simulink model "Phase6__PHASE6_ASHUGANJ_CCPP_CLOSED_LOOP_TRIP"  (R2024a)
settings: Solver=FixedStepDiscrete  StartTime=0  StopTime=0.6  FixedStep=5e-05  RelTol=1e-3
PostLoadFcn:
  | p6startupdir=fileparts(get_param(bdroot,'FileName')); while ~isfile(fullfile(p6startupdir,'scripts','setup_phase6_workspace.m')), p6startupparent=fileparts(p6startupdir); assert(~strcmp(p6startupparent,p6startupdir),'Phase6:MissingScripts','Cannot locate the Phase6 scripts folder.'); p6startupdir=p6startupparent; end; addpath(fullfile(p6startupdir,'scripts')); setup_phase6_workspace; clear p6startupdir p6startupparent;
  | phase6_color_wires(bdroot);
model workspace (MAT data in the model file):
  C.Ts = 0.001
  C.droop = 0.05
  C.governorTime_s = 0.2
  C.turbineTime_s = 0.75
  C.avrGain = 200
  C.avrTime_s = 0.02
  C.fieldMin_pu = -5
  C.fieldMax_pu = 5
  C.powerMin_pu = 0
  C.powerMax_pu = 0.982532751092
  C.pm0 = 0.786549599338
  C.vf0 = 1.78657868075
  C.vref = 1
  C.breakerDelay_s = [0.05 0.05 0.05 0.05 0.05]
  C.source = 'Phase2 canonical academic governor/AVR assumptions; LF initial state; Phase6 assumed 50 ms breaker mechanism'
  D.dc_nominal_voltage_V = 110
  D.dc_cell_count = 55
  D.dc_capacity_Ah = 200
  D.dc_internal_resistance_ohm = 0.05
  D.dc_ocv_soc = [0 1]
  D.dc_ocv_V = [105 116]
  D.dc_soc_min = 0.2
  D.dc_soc_max = 1
  D.dc_soc_initial = 1
  D.dc_cutoff_voltage_V = 105
  D.dc_max_discharge_A = 200
  D.dc_max_charge_A = 40
  D.dc_charge_efficiency = 0.9
  D.charger_nominal_voltage_V = 110
  D.charger_rated_power_kW = 20
  D.charger_unit_count = 2
  D.charger_active_units = 1
  D.charger_efficiency = 0.925
  D.charger_float_voltage_V = 123.75
  D.charger_max_current_A = 180
  D.charger_min_current_A = 0
  D.charger_response_s = 0.1
  D.charger_voltage_gain_A_per_V = 50
  D.load_relay_kW = 0.3
  D.load_control_kW = 0.5
  D.load_instrumentation_kW = 0.4
  D.load_communications_kW = 0.2
  D.load_emergency_control_kW = 0.3
  D.load_excitation_electronics_kW = 0.7
  D.load_trip_kW = 2
  D.load_trip_duration_s = 0.2
  D.load_close_kW = 3
  D.load_close_duration_s = 0.5
  D.load_emergency_additional_kW = 5
  D.continuousLoad_W = 2400
  D.acPickup_pu = 0.8
  D.serviceTolerance_W = 1e-06
  D.provenance.canonicalValues = 2
  D.provenance.continuousLoad = 2
  D.provenance.acPickup = 3
  D.provenance.brownoutLoadEquivalent = 3
  D.provenance.idealBatteryCurrentLimiter = 3
  D.provenance.serviceTolerance = 3
  D.assumptions.chargerACPickup_pu = 0.8
  D.assumptions.brownoutResistiveLoad = 1
  D.assumptions.fullSOCChargeBlocking = 1
  D.assumptions.idealBatteryCurrentLimiting = 1
  D.assumptions.proportionalUnservedLoadAllocation = 1
  D.assumptions.settledInitialCharger = 1
  P : object (value not decoded)
  Phase6BuildInfo : object (value not decoded)
  Phase6LoadFlow.model = 'PHASE6_ASHUGANJ_CCPP_DYNAMIC_MODEL'
  Phase6LoadFlow.frequency = 50
  Phase6LoadFlow.basePower = 100000000
  Phase6LoadFlow.tolerance = 1e-07
  Phase6LoadFlow.Networks.busNumber = [1 2 3 4 5 6 7 8 9 10]
  Phase6LoadFlow.Networks.SwingBus = 4
  Phase6LoadFlow.status = 1
  Phase6LoadFlow.iterations = 4
  Phase6LoadFlow.error = ''
  Phase6LoadFlow.Ybus1 = [0.0873920462832-2.08170255025i  -0.0829764098408+1.99085235815i  0+0i  0+0i  -0.000264508037957+1.56595019834e-08i  0+0i  0+0i  0+0i  -0.00011499648785-6.81612243848e-09i  0+0i; -0.0829764098316+1.99085235807i  0.162493154937-4.08162124111i  0+0i  0+0i  0+0i  -1.21290815073+1.92736685493i  0+0i  0+0i  0+0i  0+0i; 0+0i  0+0i  48400.0004643-4.58000355417e-07i  0+0i  0+0i  -48400.0000058+2.3884238942e-07i  0+0i  0+0i  0+0i  0+0i; 0+0i  0+0i  0+0i  0.00750000727735-199.185842588i  0+0i  0+0i  0+0i  0+0i  0+0i  -0.00326087287198+86.6025402558i; -0.000264500119042-5.39692317404e-11i  0+0i  -4.60726984556e-06+6.85537528968e-06i  0+0i  2645001.51335-32.1863926658i  -16.4570656799+27.6603547922i  0+0i  0+0i  -1150000.47401+1.33105697926e-05i  0+0i; 0+0i  1.06269488092+2.01409326234i  -48400.000005-9.67689493729e-06i  0+0i  15.7260334296+28.0824148285i  48400.5136015-34.5657520976i  0+0i  0+0i  0+0i  0+0i; 0+0i  0+0i  0+0i  0+0i  0+0i  0+0i  263.293444669-1351.57295033i  0+0i  -131.646722331+675.78652439i  -131.646722335+675.786524392i; 0+0i  0+0i  0+0i  0+0i  0+0i  0+0i  0+0i  263.293444769-1351.57295033i  -131.646722308+675.786524358i  -131.646722335+675.786524392i; -0.000114999950295+1.06554793283e-11i  0+0i  0+0i  0+0i  -1150000.47401+1.7196895519e-05i  7.48164142323e-07-4.6186008574e-06i  -131.646722386+675.786524482i  -131.646722309+675.78652436i  500263.499587-1351.57295615i  0+0i; 0+0i  0+0i  0+0i  -0.00326087272452+86.6025402558i  0+0i  0+0i  -131.646722334+675.786524392i  -131.646722335+675.786524392i  0+0i  263.29486254-1389.22622871i]
  Phase6LoadFlow.bus(1).handle = NaN
  Phase6LoadFlow.bus(1).ID = '*1*'
  Phase6LoadFlow.bus(1).vbase = 230000
  Phase6LoadFlow.bus(1).vref = 1
  Phase6LoadFlow.bus(1).angle = 0
  Phase6LoadFlow.bus(1).sm = []
  Phase6LoadFlow.bus(1).asm = []
  Phase6LoadFlow.bus(1).vsrc = []
  Phase6LoadFlow.bus(1).pqload = []
  Phase6LoadFlow.bus(1).rlcload = []
  Phase6LoadFlow.bus(1).blocks = 122546.00293
  Phase6LoadFlow.bus(1).busType = 'PQ'
  Phase6LoadFlow.bus(1).Sref = 0
  Phase6LoadFlow.bus(1).Vbus = 0.95508394327+0.0629961905739i
  Phase6LoadFlow.bus(1).Sbus = 1.4977567369e-17-6.86106449339e-17i
  Phase6LoadFlow.bus(1).Sgen = 0
  Phase6LoadFlow.bus(1).Spqload = -1.4977567369e-17+6.86106449339e-17i
  Phase6LoadFlow.bus(1).Sshunt = 0.00369771783189+0.0832327500202i
  Phase6LoadFlow.bus(1).Qmin = -Inf
  Phase6LoadFlow.bus(1).Qmax = Inf
  Phase6LoadFlow.bus(1).QminReached = 0
  Phase6LoadFlow.bus(1).QmaxReached = 0
  Phase6LoadFlow.bus(2).handle = NaN
  Phase6LoadFlow.bus(2).ID = '*3*'
  Phase6LoadFlow.bus(2).vbase = 6600
  Phase6LoadFlow.bus(2).vref = 1
  Phase6LoadFlow.bus(2).angle = 0
  Phase6LoadFlow.bus(2).sm = []
  Phase6LoadFlow.bus(2).asm = []
  Phase6LoadFlow.bus(2).vsrc = []
  Phase6LoadFlow.bus(2).pqload = []
  Phase6LoadFlow.bus(2).rlcload = [1 2 3]
  Phase6LoadFlow.bus(2).blocks = [123416.003784 123430.003296 123438.003418]
  Phase6LoadFlow.bus(2).busType = 'PQ'
  Phase6LoadFlow.bus(2).Sref = -0.14-0.0867642073764i
  Phase6LoadFlow.bus(2).Vbus = 0.998654558552+0.0659079236223i
  Phase6LoadFlow.bus(2).Sbus = -0.14-0.0867642073764i
  Phase6LoadFlow.bus(2).Sgen = 0
  Phase6LoadFlow.bus(2).Spqload = 0.14+0.0867642073764i
  Phase6LoadFlow.bus(2).Sshunt = -0.00722084369742-0.185139717809i
  Phase6LoadFlow.bus(2).Qmin = -Inf
  Phase6LoadFlow.bus(2).Qmax = Inf
  Phase6LoadFlow.bus(2).QminReached = 0
  Phase6LoadFlow.bus(2).QmaxReached = 0
  Phase6LoadFlow.bus(3).handle = NaN
  Phase6LoadFlow.bus(3).ID = '*4*'
  Phase6LoadFlow.bus(3).vbase = 22000
  Phase6LoadFlow.bus(3).vref = 1
  Phase6LoadFlow.bus(3).angle = 0
  Phase6LoadFlow.bus(3).sm = 1
  Phase6LoadFlow.bus(3).asm = []
  Phase6LoadFlow.bus(3).vsrc = []
  Phase6LoadFlow.bus(3).pqload = []
  Phase6LoadFlow.bus(3).rlcload = 4
  Phase6LoadFlow.bus(3).blocks = [261.009277344 5832.00402832]
  Phase6LoadFlow.bus(3).busType = 'PV'
  Phase6LoadFlow.bus(3).Sref = 3.6
  Phase6LoadFlow.bus(3).Vbus = 0.92197936676-0.387239005356i
  Phase6LoadFlow.bus(3).Sbus = 3.6+0.276166455093i
  Phase6LoadFlow.bus(3).Sgen = 3.6+0.276166455093i
  Phase6LoadFlow.bus(3).Spqload = 0
  Phase6LoadFlow.bus(3).Sshunt = 0.000458423433884+5.17701742069e-06i
  Phase6LoadFlow.bus(3).Qmin = -Inf
  Phase6LoadFlow.bus(3).Qmax = Inf
  Phase6LoadFlow.bus(3).QminReached = 0
  Phase6LoadFlow.bus(3).QmaxReached = 0
  Phase6LoadFlow.bus(4).handle = NaN
  Phase6LoadFlow.bus(4).ID = '*5*'
  Phase6LoadFlow.bus(4).vbase = 230000
  Phase6LoadFlow.bus(4).vref = 1
  Phase6LoadFlow.bus(4).angle = 0
  Phase6LoadFlow.bus(4).sm = []
  Phase6LoadFlow.bus(4).asm = []
  Phase6LoadFlow.bus(4).vsrc = 1
  Phase6LoadFlow.bus(4).pqload = []
  Phase6LoadFlow.bus(4).rlcload = []
  Phase6LoadFlow.bus(4).blocks = 121606.003174
  Phase6LoadFlow.bus(4).busType = 'swing'
  Phase6LoadFlow.bus(4).Sref = 0
  Phase6LoadFlow.bus(4).Vbus = 1
  Phase6LoadFlow.bus(4).Sbus = -3.45133752941+0.264692642147i
  Phase6LoadFlow.bus(4).Sgen = -3.45133752941+0.264692642147i
  Phase6LoadFlow.bus(4).Spqload = 0
  Phase6LoadFlow.bus(4).Sshunt = 0.00423913447911+112.583302333i
  Phase6LoadFlow.bus(4).Qmin = -Inf
  Phase6LoadFlow.bus(4).Qmax = Inf
  Phase6LoadFlow.bus(4).QminReached = 0
  Phase6LoadFlow.bus(4).QmaxReached = 0
  Phase6LoadFlow.bus(5).handle = NaN
  Phase6LoadFlow.bus(5).ID = '*6*'
  Phase6LoadFlow.bus(5).vbase = 230000
  Phase6LoadFlow.bus(5).vref = 1
  Phase6LoadFlow.bus(5).angle = 0
  Phase6LoadFlow.bus(5).sm = []
  Phase6LoadFlow.bus(5).asm = []
  Phase6LoadFlow.bus(5).vsrc = []
  Phase6LoadFlow.bus(5).pqload = []
  Phase6LoadFlow.bus(5).rlcload = []
  Phase6LoadFlow.bus(5).blocks = 1170.01000977
  Phase6LoadFlow.bus(5).busType = 'PQ'
  Phase6LoadFlow.bus(5).Sref = 0
  Phase6LoadFlow.bus(5).Vbus = 0.998782663812+0.0182714556672i
  Phase6LoadFlow.bus(5).Sbus = 4.64828536298e-10+2.30425102224e-11i
  Phase6LoadFlow.bus(5).Sgen = 0
  Phase6LoadFlow.bus(5).Spqload = -4.64828536298e-10-2.30425102224e-11i
  Phase6LoadFlow.bus(5).Sshunt = 1491862.09587+0.00326094848941i
  Phase6LoadFlow.bus(5).Qmin = -Inf
  Phase6LoadFlow.bus(5).Qmax = Inf
  Phase6LoadFlow.bus(5).QminReached = 0
  Phase6LoadFlow.bus(5).QmaxReached = 0
  Phase6LoadFlow.bus(6).handle = NaN
  Phase6LoadFlow.bus(6).ID = '*8*'
  Phase6LoadFlow.bus(6).vbase = 22000
  Phase6LoadFlow.bus(6).vref = 1
  Phase6LoadFlow.bus(6).angle = 0
  Phase6LoadFlow.bus(6).sm = []
  Phase6LoadFlow.bus(6).asm = []
  Phase6LoadFlow.bus(6).vsrc = []
  Phase6LoadFlow.bus(6).pqload = []
  Phase6LoadFlow.bus(6).rlcload = []
  Phase6LoadFlow.bus(6).blocks = 122360.003052
  Phase6LoadFlow.bus(6).busType = 'PQ'
  Phase6LoadFlow.bus(6).Sref = 0
  Phase6LoadFlow.bus(6).Vbus = 0.921913008067-0.387204945387i
  Phase6LoadFlow.bus(6).Sbus = 8.11644335598e-12+5.36613214691e-13i
  Phase6LoadFlow.bus(6).Sgen = 0
  Phase6LoadFlow.bus(6).Spqload = -8.11644335598e-12-5.36613214691e-13i
  Phase6LoadFlow.bus(6).Sshunt = 0.00480844142117+0.107036142686i
  Phase6LoadFlow.bus(6).Qmin = -Inf
  Phase6LoadFlow.bus(6).Qmax = Inf
  Phase6LoadFlow.bus(6).QminReached = 0
  Phase6LoadFlow.bus(6).QmaxReached = 0
  Phase6LoadFlow.bus(7).handle = NaN
  Phase6LoadFlow.bus(7).ID = '*9*'
  Phase6LoadFlow.bus(7).vbase = 100000
  Phase6LoadFlow.bus(7).vref = 1
  Phase6LoadFlow.bus(7).angle = 0
  Phase6LoadFlow.bus(7).sm = []
  Phase6LoadFlow.bus(7).asm = []
  Phase6LoadFlow.bus(7).vsrc = []
  Phase6LoadFlow.bus(7).pqload = []
  Phase6LoadFlow.bus(7).rlcload = []
  Phase6LoadFlow.bus(7).blocks = 121211.00293
  Phase6LoadFlow.bus(7).busType = 'PQ'
  Phase6LoadFlow.bus(7).Sref = 0
  Phase6LoadFlow.bus(7).Vbus = 2.29707127118+0.0409383935568i
  Phase6LoadFlow.bus(7).Sbus = 5.31601850694e-13-5.12985224674e-13i
  Phase6LoadFlow.bus(7).Sgen = 0
  Phase6LoadFlow.bus(7).Spqload = -5.31601850694e-13+5.12985224674e-13i
  Phase6LoadFlow.bus(7).Sshunt = -7.7574979931e-08-0.000519611737109i
  Phase6LoadFlow.bus(7).Qmin = -Inf
  Phase6LoadFlow.bus(7).Qmax = Inf
  Phase6LoadFlow.bus(7).QminReached = 0
  Phase6LoadFlow.bus(7).QmaxReached = 0
  Phase6LoadFlow.bus(8).handle = NaN
  Phase6LoadFlow.bus(8).ID = '*10*'
  Phase6LoadFlow.bus(8).vbase = 100000
  Phase6LoadFlow.bus(8).vref = 1
  Phase6LoadFlow.bus(8).angle = 0
  Phase6LoadFlow.bus(8).sm = []
  Phase6LoadFlow.bus(8).asm = []
  Phase6LoadFlow.bus(8).vsrc = []
  Phase6LoadFlow.bus(8).pqload = []
  Phase6LoadFlow.bus(8).rlcload = []
  Phase6LoadFlow.bus(8).blocks = 120500.003662
  Phase6LoadFlow.bus(8).busType = 'PQ'
  Phase6LoadFlow.bus(8).Sref = 0
  Phase6LoadFlow.bus(8).Vbus = 2.29707127109+0.0409383933626i
  Phase6LoadFlow.bus(8).Sbus = -2.33221829935e-13-1.57153476947e-12i
  Phase6LoadFlow.bus(8).Sgen = 0
  Phase6LoadFlow.bus(8).Spqload = 2.33221829935e-13+1.57153476947e-12i
  Phase6LoadFlow.bus(8).Sshunt = 6.68020889729e-07-0.000519459230386i
  Phase6LoadFlow.bus(8).Qmin = -Inf
  Phase6LoadFlow.bus(8).Qmax = Inf
  Phase6LoadFlow.bus(8).QminReached = 0
  Phase6LoadFlow.bus(8).QmaxReached = 0
  Phase6LoadFlow.bus(9).handle = NaN
  Phase6LoadFlow.bus(9).ID = '*11*'
  Phase6LoadFlow.bus(9).vbase = 100000
  Phase6LoadFlow.bus(9).vref = 1
  Phase6LoadFlow.bus(9).angle = 0
  Phase6LoadFlow.bus(9).sm = []
  Phase6LoadFlow.bus(9).asm = []
  Phase6LoadFlow.bus(9).vsrc = []
  Phase6LoadFlow.bus(9).pqload = []
  Phase6LoadFlow.bus(9).rlcload = []
  Phase6LoadFlow.bus(9).blocks = 120500.003662
  Phase6LoadFlow.bus(9).busType = 'PQ'
  Phase6LoadFlow.bus(9).Sref = 0
  Phase6LoadFlow.bus(9).Vbus = 2.29719712563+0.0420241160697i
  Phase6LoadFlow.bus(9).Sbus = -5.34705002516e-10-1.81416564522e-11i
  Phase6LoadFlow.bus(9).Sgen = 0
  Phase6LoadFlow.bus(9).Spqload = 5.34705002516e-10+1.81416564522e-11i
  Phase6LoadFlow.bus(9).Sshunt = -3431273.84385-0.000545427580754i
  Phase6LoadFlow.bus(9).Qmin = -Inf
  Phase6LoadFlow.bus(9).Qmax = Inf
  Phase6LoadFlow.bus(9).QminReached = 0
  Phase6LoadFlow.bus(9).QmaxReached = 0
  Phase6LoadFlow.bus(10).handle = NaN
  Phase6LoadFlow.bus(10).ID = '*12*'
  Phase6LoadFlow.bus(10).vbase = 100000
  Phase6LoadFlow.bus(10).vref = 1
  Phase6LoadFlow.bus(10).angle = 0
  Phase6LoadFlow.bus(10).sm = []
  Phase6LoadFlow.bus(10).asm = []
  Phase6LoadFlow.bus(10).vsrc = []
  Phase6LoadFlow.bus(10).pqload = []
  Phase6LoadFlow.bus(10).rlcload = []
  Phase6LoadFlow.bus(10).blocks = 120508.003296
  Phase6LoadFlow.bus(10).busType = 'PQ'
  Phase6LoadFlow.bus(10).Sref = 0
  Phase6LoadFlow.bus(10).Vbus = 2.29694509322+0.0398527281134i
  Phase6LoadFlow.bus(10).Sbus = 2.61132424068e-12+4.5307306338e-14i
  Phase6LoadFlow.bus(10).Sgen = 0
  Phase6LoadFlow.bus(10).Spqload = -2.61132424068e-12-4.5307306338e-14i
  Phase6LoadFlow.bus(10).Sshunt = -0.00972652684513-258.332451941i
  Phase6LoadFlow.bus(10).Qmin = -Inf
  Phase6LoadFlow.bus(10).Qmax = Inf
  Phase6LoadFlow.bus(10).QminReached = 0
  Phase6LoadFlow.bus(10).QmaxReached = 0
  Phase6LoadFlow.sm.handle = 261.009277344
  Phase6LoadFlow.sm.busNumber = 3
  Phase6LoadFlow.sm.busID = '*4*'
  Phase6LoadFlow.sm.generatorType = 'PV'
  Phase6LoadFlow.sm.Pnom = 458000000
  Phase6LoadFlow.sm.Vnom = 22000
  Phase6LoadFlow.sm.P = 360000000
  Phase6LoadFlow.sm.Q = 0
  Phase6LoadFlow.sm.Qmin = -Inf
  Phase6LoadFlow.sm.Qmax = Inf
  Phase6LoadFlow.sm.S = 3.6+0.276166455093i
  Phase6LoadFlow.sm.I = 0.701350064837-0.359973841194i
  Phase6LoadFlow.sm.Pmec = 360239716.497
  Phase6LoadFlow.sm.Vt = 0.92197936676-0.387239005356i
  Phase6LoadFlow.sm.Vf = 1.78657868075
  Phase6LoadFlow.sm.th0 = -61.5748702309
  Phase6LoadFlow.sm.dw0 = 0
  Phase6LoadFlow.asm = []
  Phase6LoadFlow.vsrc.handle = 121606.003174
  Phase6LoadFlow.vsrc.busNumber = 4
  Phase6LoadFlow.vsrc.busID = '*5*'
  Phase6LoadFlow.vsrc.generatorType = 'swing'
  Phase6LoadFlow.vsrc.Vnom = 230000
  Phase6LoadFlow.vsrc.P = 10000
  Phase6LoadFlow.vsrc.Q = 0
  Phase6LoadFlow.vsrc.Qmin = -Inf
  Phase6LoadFlow.vsrc.Qmax = Inf
  Phase6LoadFlow.vsrc.S = -3.45133752941+0.264692642147i
  Phase6LoadFlow.vsrc.I = -3.45133752941-0.264692642147i
  Phase6LoadFlow.vsrc.Vt = 1
  Phase6LoadFlow.vsrc.Vint = 1
  Phase6LoadFlow.pqload = []
  Phase6LoadFlow.rlcload(1).handle = 123416.003784
  Phase6LoadFlow.rlcload(1).busNumber = 2
  Phase6LoadFlow.rlcload(1).busID = '*3*'
  Phase6LoadFlow.rlcload(1).loadType = 'PQ'
  Phase6LoadFlow.rlcload(1).Vnom = 6600
  Phase6LoadFlow.rlcload(1).P = 9017793.59431
  Phase6LoadFlow.rlcload(1).Q = 5588726.52496
  Phase6LoadFlow.rlcload(1).S = 0.0901779359431+0.0558872652496i
  Phase6LoadFlow.rlcload(1).I = 0.0935851574128-0.049786246322i
  Phase6LoadFlow.rlcload(1).Vt = 0.998654558552+0.0659079236223i
  Phase6LoadFlow.rlcload(2).handle = 123430.003296
  Phase6LoadFlow.rlcload(2).busNumber = 2
  Phase6LoadFlow.rlcload(2).busID = '*3*'
  Phase6LoadFlow.rlcload(2).loadType = 'PQ'
  Phase6LoadFlow.rlcload(2).Vnom = 6600
  Phase6LoadFlow.rlcload(2).P = 2491103.20285
  Phase6LoadFlow.rlcload(2).Q = 1543847.10634
  Phase6LoadFlow.rlcload(2).S = 0.0249110320285+0.0154384710634i
  Phase6LoadFlow.rlcload(2).I = 0.0258522534289-0.0137531067188i
  Phase6LoadFlow.rlcload(2).Vt = 0.998654558552+0.0659079236223i
  Phase6LoadFlow.rlcload(3).handle = 123438.003418
  Phase6LoadFlow.rlcload(3).busNumber = 2
  Phase6LoadFlow.rlcload(3).busID = '*3*'
  Phase6LoadFlow.rlcload(3).loadType = 'PQ'
  Phase6LoadFlow.rlcload(3).Vnom = 6600
  Phase6LoadFlow.rlcload(3).P = 2491103.20285
  Phase6LoadFlow.rlcload(3).Q = 1543847.10634
  Phase6LoadFlow.rlcload(3).S = 0.0249110320285+0.0154384710634i
  Phase6LoadFlow.rlcload(3).I = 0.0258522534289-0.0137531067188i
  Phase6LoadFlow.rlcload(3).Vt = 0.998654558552+0.0659079236223i
  Phase6LoadFlow.rlcload(4).handle = 5832.00402832
  Phase6LoadFlow.rlcload(4).busNumber = 3
  Phase6LoadFlow.rlcload(4).busID = '*4*'
  Phase6LoadFlow.rlcload(4).loadType = 'Z'
  Phase6LoadFlow.rlcload(4).Vnom = 22000
  Phase6LoadFlow.rlcload(4).P = 10
  Phase6LoadFlow.rlcload(4).Q = 0
  Phase6LoadFlow.rlcload(4).S = 1e-07
  Phase6LoadFlow.rlcload(4).I = 0
  Phase6LoadFlow.rlcload(4).Vt = 0.92197936676-0.387239005356i
  Phase6LoadFlow.LoadFlowSolver = 'PositiveSequence'
  Phase6Metadata.parameters.Ts = 0.001
  Phase6Metadata.parameters.droop = 0.05
  Phase6Metadata.parameters.governorTime_s = 0.2
  Phase6Metadata.parameters.turbineTime_s = 0.75
  Phase6Metadata.parameters.avrGain = 200
  Phase6Metadata.parameters.avrTime_s = 0.02
  Phase6Metadata.parameters.fieldMin_pu = -5
  Phase6Metadata.parameters.fieldMax_pu = 5
  Phase6Metadata.parameters.powerMin_pu = 0
  Phase6Metadata.parameters.powerMax_pu = 0.982532751092
  Phase6Metadata.parameters.pm0 = 0.786549599338
  Phase6Metadata.parameters.vf0 = 1.78657868075
  Phase6Metadata.parameters.vref = 1
  Phase6Metadata.parameters.breakerDelay_s = [0.05 0.05 0.05 0.05 0.05]
  Phase6Metadata.parameters.source = 'Phase2 canonical academic governor/AVR assumptions; LF initial state; Phase6 assumed 50 ms breaker mechanism'
  Phase6Metadata.relayParameters.settingValues = [17170.8  1.14472  15000  0.1  NaN  NaN; 4  0.2  20  0.15  NaN  NaN; 1380  0.8625  1600  0.55  NaN  NaN; 1500  0.9375  1600  0.8  NaN  NaN; 17171  1.14473333333  15000  NaN  3  NaN; 2403.8  0.160253333333  15000  NaN  NaN  0.045; 387.84  0.2424  1600  NaN  NaN  0.045; 320  0.2  1600  NaN  NaN  0.035; 320  0.2  1600  NaN  0.05  0.035]
  Phase6Metadata.relayParameters.settingSourceRows = [1 2 3 4 5 6 7 8 9]
  Phase6Metadata.relayParameters.pickup_A = [17170.8 1380 4 2403.8 387.84 320 320]
  Phase6Metadata.relayParameters.pickupSecondary_A = [1.14472 0.8625 0.2 0.160253333333 0.2424 0.2 0.2]
  Phase6Metadata.relayParameters.ctRatio = [15000 1600 20 15000 1600 1600 1600]
  Phase6Metadata.relayParameters.tms = [0.1 0.55 0.15]
  Phase6Metadata.relayParameters.delay_s = [0.045 0.045 0.035 0.035]
  Phase6Metadata.relayParameters.lvToHv = 0.095652173913
  Phase6Metadata.relayParameters.iecK = 0.14
  Phase6Metadata.relayParameters.iecAlpha = 0.02
  Phase6Metadata.relayParameters.highsetEnabled = [0 0 0 0 0 0 0]
  Phase6Metadata.relayParameters.slope1 = [0.3 0.3 0.3 0.3]
  Phase6Metadata.relayParameters.slope2 = [0.3 0.6 0.3 0.3]
  Phase6Metadata.relayParameters.knee_A = [12019 2585.6 1600 1600]
  Phase6Metadata.relayParameters.restraintFactor = 0.5
  Phase6Metadata.relayParameters.lineSchemeClearingProxy_s = 0.05
  Phase6Metadata.relayParameters.phase5.GEN_S_MVA = 458
  Phase6Metadata.relayParameters.phase5.GEN_V_kV = 22
  Phase6Metadata.relayParameters.phase5.GEN_rated_A = 12019
  Phase6Metadata.relayParameters.phase5.GEN_maximum_operating_A = 14309
  Phase6Metadata.relayParameters.phase5.GEN_phase_CT = 15000
  Phase6Metadata.relayParameters.phase5.GEN_51_pickup_A = 17170.8
  Phase6Metadata.relayParameters.phase5.GEN_51_secondary_A = 1.14472
  Phase6Metadata.relayParameters.phase5.GEN_51_TMS = 0.1
  Phase6Metadata.relayParameters.phase5.GEN_51N_CT = 20
  Phase6Metadata.relayParameters.phase5.GEN_51N_secondary_A = 0.2
  Phase6Metadata.relayParameters.phase5.GEN_51N_pickup_A = 4
  Phase6Metadata.relayParameters.phase5.GEN_51N_TMS = 0.15
  Phase6Metadata.relayParameters.phase5.GEN_87G_pu = 0.2
  Phase6Metadata.relayParameters.phase5.GEN_87G_pickup_A = 2403.8
  Phase6Metadata.relayParameters.phase5.GEN_87G_highset_enabled = 0
  Phase6Metadata.relayParameters.phase5.GEN_87G_time_s = 0.045
  Phase6Metadata.relayParameters.phase5.GEN_Xdpp_sat_pu = 0.2248
  Phase6Metadata.relayParameters.phase5.GEN_Xdpp_unsat_pu = 0.2608
  Phase6Metadata.relayParameters.phase5.GEN_X2_pu = 0.2242
  Phase6Metadata.relayParameters.phase5.GEN_X0_pu = 0.128
  Phase6Metadata.relayParameters.phase5.GEN_Ra_ohm = 0.00089
  Phase6Metadata.relayParameters.phase5.GEN_R1_pu = 0.000842190082645
  Phase6Metadata.relayParameters.phase5.GEN_R2_pu = 0.000842190082645
  Phase6Metadata.relayParameters.phase5.GEN_R0_pu = 0.00126328512397
  Phase6Metadata.relayParameters.phase5.GSUT_S_MVA = 515
  Phase6Metadata.relayParameters.phase5.GSUT_HV_kV = 230
  Phase6Metadata.relayParameters.phase5.GSUT_LV_kV = 22
  Phase6Metadata.relayParameters.phase5.GSUT_rated_exact_A = 1292.76255927
  Phase6Metadata.relayParameters.phase5.GSUT_rated_A = 1292.8
  Phase6Metadata.relayParameters.phase5.GSUT_maximum_load_anchor_A = 1149.68010126
  Phase6Metadata.relayParameters.phase5.GSUT_CT = 1600
  Phase6Metadata.relayParameters.phase5.GSUT_documentary_CT = 1500
  Phase6Metadata.relayParameters.phase5.GSUT_51_pickup_A = 1380
  Phase6Metadata.relayParameters.phase5.GSUT_51_secondary_A = 0.8625
  Phase6Metadata.relayParameters.phase5.GSUT_51_TMS = 0.55
  Phase6Metadata.relayParameters.phase5.GSUT_87T_pu = 0.3
  Phase6Metadata.relayParameters.phase5.GSUT_87T_pickup_A = 387.84
  Phase6Metadata.relayParameters.phase5.GSUT_87T_slope1_percent = 30
  Phase6Metadata.relayParameters.phase5.GSUT_87T_slope2_percent = 60
  Phase6Metadata.relayParameters.phase5.GSUT_87T_time_s = 0.045
  Phase6Metadata.relayParameters.phase5.GSUT_Z1_pu = 0.1663
  Phase6Metadata.relayParameters.phase5.GSUT_copper_loss_MW = 0.9122
  Phase6Metadata.relayParameters.phase5.GSUT_OEM_Z1_pu = 0.16
  Phase6Metadata.relayParameters.phase5.GSUT_OEM_copper_loss_MW = 1.095
  Phase6Metadata.relayParameters.phase5.GSUT_R1_pu = 0.00177126213592
  Phase6Metadata.relayParameters.phase5.GSUT_X1_pu = 0.166290566872
  Phase6Metadata.relayParameters.phase5.GSUT_vector_clock = 1
  Phase6Metadata.relayParameters.phase5.GSUT_HV_solid_grounded = 1
  Phase6Metadata.relayParameters.phase5.Q0_CT = 1600
  Phase6Metadata.relayParameters.phase5.Q0_51_pickup_A = 1500
  Phase6Metadata.relayParameters.phase5.Q0_51_secondary_A = 0.9375
  Phase6Metadata.relayParameters.phase5.Q0_51_TMS = 0.8
  Phase6Metadata.relayParameters.phase5.Q0_continuous_A = 2000
  Phase6Metadata.relayParameters.phase5.Q0_interrupting_kA = 50
  Phase6Metadata.relayParameters.phase5.Q0_making_kA = 125
  Phase6Metadata.relayParameters.phase5.Q0_shortcircuit_s = 3
  Phase6Metadata.relayParameters.phase5.BUS_87B_pu = 0.2
  Phase6Metadata.relayParameters.phase5.BUS_87B_base_A = 1600
  Phase6Metadata.relayParameters.phase5.BUS_87B_pickup_A = 320
  Phase6Metadata.relayParameters.phase5.BUS_87B_slope_percent = 30
  Phase6Metadata.relayParameters.phase5.BUS_87B_time_s = 0.035
  Phase6Metadata.relayParameters.phase5.LINE_87L_pu = 0.2
  Phase6Metadata.relayParameters.phase5.LINE_87L_base_A = 1600
  Phase6Metadata.relayParameters.phase5.LINE_87L_pickup_A = 320
  Phase6Metadata.relayParameters.phase5.LINE_87L_time_s = 0.035
  Phase6Metadata.relayParameters.phase5.LINE_87L_clearing_s = 0.05
  Phase6Metadata.relayParameters.phase5.BF_230kV_s = 0.15
  Phase6Metadata.relayParameters.phase5.BF_22kV_s = 0.12
  Phase6Metadata.relayParameters.phase5.CTI_s = 0.3
  Phase6Metadata.relayParameters.phase5.GEN_64G_U20min_V = 1
  Phase6Metadata.relayParameters.phase5.GEN_64G_I20min_A = 0.01
  Phase6Metadata.relayParameters.phase5.GEN_64G_trip_R_ohm = 20
  Phase6Metadata.relayParameters.phase5.GEN_64G_alarm_R_ohm = 100
  Phase6Metadata.relayParameters.phase5.GEN_64G_trip_delay_s = 1
  Phase6Metadata.relayParameters.phase5.GEN_64G_alarm_delay_s = 10
  Phase6Metadata.relayParameters.phase5.GEN_64G_correction_angle_deg = 0
  Phase6Metadata.relayParameters.phase5.NER_R_ohm = 60
  Phase6Metadata.relayParameters.phase5.NER_rating_kVA = 135
  Phase6Metadata.relayParameters.phase5.NER_duration_s = 20
  Phase6Metadata.relayParameters.phase5.NER_primary_kV = 12.7017059222
  Phase6Metadata.relayParameters.phase5.NER_secondary_V = 500
  Phase6Metadata.relayParameters.phase5.NGT_ratio = 25.4034118443
  Phase6Metadata.relayParameters.phase5.NER_loading_LV_ohm = 2.62
  Phase6Metadata.relayParameters.phase5.NER_effective_HV_ohm = 1750.77333333
  Phase6Metadata.relayParameters.phase5.SOUTH_length_km = 0.7
  Phase6Metadata.relayParameters.phase5.SOUTH_circuits = 2
  Phase6Metadata.relayParameters.phase5.SOUTH_R1_per_km = 0.08
  Phase6Metadata.relayParameters.phase5.SOUTH_R1_total_ohm = 0.056
  Phase6Metadata.relayParameters.phase5.SOUTH_X1_per_km = 0.35
  Phase6Metadata.relayParameters.phase5.SOUTH_X1_total_ohm = 0.245
  Phase6Metadata.relayParameters.phase5.SOUTH_B1_per_km = 4.2
  Phase6Metadata.relayParameters.phase5.SOUTH_B1_total_uS = 2.94
  Phase6Metadata.relayParameters.phase5.SOUTH_R0_per_km = 0.25
  Phase6Metadata.relayParameters.phase5.SOUTH_R0_total_ohm = 0.175
  Phase6Metadata.relayParameters.phase5.SOUTH_X0_per_km = 1.2
  Phase6Metadata.relayParameters.phase5.SOUTH_X0_total_ohm = 0.84
  Phase6Metadata.relayParameters.phase5.SOUTH_B0_per_km = 2.8
  Phase6Metadata.relayParameters.phase5.SOUTH_B0_total_uS = 1.96
  Phase6Metadata.relayParameters.phase5.DIST21_zone1_fraction = 0.8
  Phase6Metadata.relayParameters.phase5.DIST21_zone1_R_ohm = 0.0448
  Phase6Metadata.relayParameters.phase5.DIST21_zone1_X_ohm = 0.196
  Phase6Metadata.relayParameters.phase5.DIST21_zone1_time_s = 0
  Phase6Metadata.relayParameters.phase5.DIST21_zone2_fraction = 1.2
  Phase6Metadata.relayParameters.phase5.DIST21_zone2_R_ohm = 0.0672
  Phase6Metadata.relayParameters.phase5.DIST21_zone2_X_ohm = 0.294
  Phase6Metadata.relayParameters.phase5.DIST21_zone2_time_s = 0.3
  Phase6Metadata.relayParameters.phase5.DIST21_zone3_fraction = 2
  Phase6Metadata.relayParameters.phase5.DIST21_zone3_R_ohm = 0.112
  Phase6Metadata.relayParameters.phase5.DIST21_zone3_X_ohm = 0.49
  Phase6Metadata.relayParameters.phase5.DIST21_zone3_time_s = 0.8
  Phase6Metadata.relayParameters.phase5.NORTH_BHULTA_length_km = 69
  Phase6Metadata.relayParameters.phase5.NORTH_BHULTA_circuits = 2
  Phase6Metadata.relayParameters.phase5.NORTH_BHULTA_voltage_kV = 400
  Phase6Metadata.relayParameters.phase5.NORTH_BHULTA_R1_ohm_per_km = 0.031
  Phase6Metadata.relayParameters.phase5.NORTH_BHULTA_R1_total_ohm = 2.139
  Phase6Metadata.relayParameters.phase5.NORTH_BHULTA_X1_ohm_per_km = 0.32
  Phase6Metadata.relayParameters.phase5.NORTH_BHULTA_X1_total_ohm = 22.08
  Phase6Metadata.relayParameters.phase5.NORTH_BHULTA_R0_ohm_per_km = 0.28
  Phase6Metadata.relayParameters.phase5.NORTH_BHULTA_R0_total_ohm = 19.32
  Phase6Metadata.relayParameters.phase5.NORTH_BHULTA_X0_ohm_per_km = 1.15
  Phase6Metadata.relayParameters.phase5.NORTH_BHULTA_X0_total_ohm = 79.35
  Phase6Metadata.relayParameters.phase5.GHORASAL_ASHUGANJ_230_length_km = 44
  Phase6Metadata.relayParameters.phase5.GHORASAL_ASHUGANJ_230_circuits = 2
  Phase6Metadata.relayParameters.phase5.GHORASAL_ASHUGANJ_230_voltage_kV = 230
  Phase6Metadata.relayParameters.phase5.GHORASAL_ASHUGANJ_230_R1_ohm_per_km = 0.0855
  Phase6Metadata.relayParameters.phase5.GHORASAL_ASHUGANJ_230_R1_total_ohm = 3.762
  Phase6Metadata.relayParameters.phase5.GHORASAL_ASHUGANJ_230_X1_ohm_per_km = 0.4
  Phase6Metadata.relayParameters.phase5.GHORASAL_ASHUGANJ_230_X1_total_ohm = 17.6
  Phase6Metadata.relayParameters.phase5.GHORASAL_ASHUGANJ_230_R0_ohm_per_km = 0.25
  Phase6Metadata.relayParameters.phase5.GHORASAL_ASHUGANJ_230_R0_total_ohm = 11
  Phase6Metadata.relayParameters.phase5.GHORASAL_ASHUGANJ_230_X0_ohm_per_km = 1.45
  Phase6Metadata.relayParameters.phase5.GHORASAL_ASHUGANJ_230_X0_total_ohm = 63.8
  Phase6Metadata.relayParameters.phase5.ASHUGANJ_COMILLA_NORTH_length_km = 79
  Phase6Metadata.relayParameters.phase5.ASHUGANJ_COMILLA_NORTH_circuits = 2
  Phase6Metadata.relayParameters.phase5.ASHUGANJ_COMILLA_NORTH_voltage_kV = 230
  Phase6Metadata.relayParameters.phase5.ASHUGANJ_COMILLA_NORTH_R1_ohm_per_km = 0.062
  Phase6Metadata.relayParameters.phase5.ASHUGANJ_COMILLA_NORTH_R1_total_ohm = 4.898
  Phase6Metadata.relayParameters.phase5.ASHUGANJ_COMILLA_NORTH_X1_ohm_per_km = 0.4
  Phase6Metadata.relayParameters.phase5.ASHUGANJ_COMILLA_NORTH_X1_total_ohm = 31.6
  Phase6Metadata.relayParameters.phase5.ASHUGANJ_COMILLA_NORTH_R0_ohm_per_km = 0.25
  Phase6Metadata.relayParameters.phase5.ASHUGANJ_COMILLA_NORTH_R0_total_ohm = 19.75
  Phase6Metadata.relayParameters.phase5.ASHUGANJ_COMILLA_NORTH_X0_ohm_per_km = 1.45
  Phase6Metadata.relayParameters.phase5.ASHUGANJ_COMILLA_NORTH_X0_total_ohm = 114.55
  Phase6Metadata.relayParameters.phase5.ASHUGANJ_SIRAJGANJ_length_km = 144
  Phase6Metadata.relayParameters.phase5.ASHUGANJ_SIRAJGANJ_circuits = 2
  Phase6Metadata.relayParameters.phase5.ASHUGANJ_SIRAJGANJ_voltage_kV = 230
  Phase6Metadata.relayParameters.phase5.ASHUGANJ_SIRAJGANJ_R1_ohm_per_km = 0.065
  Phase6Metadata.relayParameters.phase5.ASHUGANJ_SIRAJGANJ_R1_total_ohm = 9.36
  Phase6Metadata.relayParameters.phase5.ASHUGANJ_SIRAJGANJ_X1_ohm_per_km = 0.34
  Phase6Metadata.relayParameters.phase5.ASHUGANJ_SIRAJGANJ_X1_total_ohm = 48.96
  Phase6Metadata.relayParameters.phase5.ASHUGANJ_SIRAJGANJ_R0_ohm_per_km = 0.24
  Phase6Metadata.relayParameters.phase5.ASHUGANJ_SIRAJGANJ_R0_total_ohm = 34.56
  Phase6Metadata.relayParameters.phase5.ASHUGANJ_SIRAJGANJ_X0_ohm_per_km = 1.25
  Phase6Metadata.relayParameters.phase5.ASHUGANJ_SIRAJGANJ_X0_total_ohm = 180
  Phase6Metadata.relayParameters.phase5.ASHUGANJ_KISHOREGANJ_length_km = 52
  Phase6Metadata.relayParameters.phase5.ASHUGANJ_KISHOREGANJ_circuits = 2
  Phase6Metadata.relayParameters.phase5.ASHUGANJ_KISHOREGANJ_voltage_kV = 132
  Phase6Metadata.relayParameters.phase5.ASHUGANJ_KISHOREGANJ_R1_ohm_per_km = 0.083
  Phase6Metadata.relayParameters.phase5.ASHUGANJ_KISHOREGANJ_R1_total_ohm = 4.316
  Phase6Metadata.relayParameters.phase5.ASHUGANJ_KISHOREGANJ_X1_ohm_per_km = 0.38
  Phase6Metadata.relayParameters.phase5.ASHUGANJ_KISHOREGANJ_X1_total_ohm = 19.76
  Phase6Metadata.relayParameters.phase5.ASHUGANJ_KISHOREGANJ_R0_ohm_per_km = 0.25
  Phase6Metadata.relayParameters.phase5.ASHUGANJ_KISHOREGANJ_R0_total_ohm = 13
  Phase6Metadata.relayParameters.phase5.ASHUGANJ_KISHOREGANJ_X0_ohm_per_km = 1.45
  Phase6Metadata.relayParameters.phase5.ASHUGANJ_KISHOREGANJ_X0_total_ohm = 75.4
  Phase6Metadata.relayParameters.phase5.GRID_Isc_kA = 45.01
  Phase6Metadata.relayParameters.phase5.GRID_XR = 10.99
  Phase6Metadata.relayParameters.phase5.GRID_Zth_ohm = 2.95024576569
  Phase6Metadata.relayParameters.phase5.GRID_Rth_ohm = 0.267343748148
  Phase6Metadata.relayParameters.phase5.GRID_Xth_ohm = 2.93810779215
  Phase6Metadata.relayParameters.phase5.GRID_Ssc_GVA = 17.9307095752
  Phase6Metadata.relayParameters.phase5.GRID_reported_Z_ohm = 3.25
  Phase6Metadata.relayParameters.phase5.GRID_Z2_Z1_ratio = 1
  Phase6Metadata.relayParameters.phase5.GRID_Z0_Z1_ratio = 3
  Phase6Metadata.relayParameters.phase5.GRID_R2_ohm = 0.267343748148
  Phase6Metadata.relayParameters.phase5.GRID_X2_ohm = 2.93810779215
  Phase6Metadata.relayParameters.phase5.GRID_R0_ohm = 0.802031244445
  Phase6Metadata.relayParameters.phase5.GRID_X0_ohm = 8.81432337645
  Phase6Metadata.relayParameters.phase5.MOTOR_P_MW = 12
  Phase6Metadata.relayParameters.phase5.MOTOR_Q_Mvar = 5
  Phase6Metadata.relayParameters.phase5.MOTOR_MV_P_MW = 9
  Phase6Metadata.relayParameters.phase5.MOTOR_LV_P_MW = 3
  Phase6Metadata.relayParameters.phase5.MOTOR_MV_V_kV = 6.6
  Phase6Metadata.relayParameters.phase5.MOTOR_LV_V_kV = 0.4
  Phase6Metadata.relayParameters.phase5.MOTOR_ILR_Ir = 5
  Phase6Metadata.relayParameters.phase5.CT_accuracy_limit_factor = 20
  Phase6Metadata.relayParameters.phase5.CT_accuracy_boundary_A = 32000
  Phase6Metadata.relayParameters.phase5.CT_above_boundary_transfer = 0.75
  Phase6Metadata.relayParameters.provenance.settings = 2
  Phase6Metadata.relayParameters.provenance.parameters = 2
  Phase6Metadata.relayParameters.provenance.pickup = [2 2 2 2 2 2 2]
  Phase6Metadata.relayParameters.provenance.tms = [2 2 2]
  Phase6Metadata.relayParameters.provenance.delay = [2 2 2 2]
  Phase6Metadata.relayParameters.provenance.lvToHv = 2
  Phase6Metadata.relayParameters.provenance.slope1 = [3 2 2 3]
  Phase6Metadata.relayParameters.provenance.slope2 = [3 2 2 3]
  Phase6Metadata.relayParameters.provenance.knee = [3 3 3 3]
  Phase6Metadata.relayParameters.provenance.restraintFactor = 3
  Phase6Metadata.relayParameters.provenance.characteristic = 3
  Phase6Metadata.relayParameters.assumptions.generatorBias_percent = 30
  Phase6Metadata.relayParameters.assumptions.lineBias_percent = 30
  Phase6Metadata.relayParameters.assumptions.transformerKneeRatedMultiple = 2
  Phase6Metadata.relayParameters.assumptions.halfSumRestraint = 1
  Phase6Metadata.relayParameters.assumptions.idealSynchronizedPhasors = 1
  Phase6Metadata.relayParameters.assumptions.communicationDelay_s = 0
  Phase6Metadata.relayParameters.assumptions.harmonicBlockingImplemented = 0
  Phase6Metadata.relayParameters.assumptions.ctSaturationImplemented = 0
  Phase6Metadata.measurements = 'PHASE6_ASHUGANJ_CCPP_DYNAMIC_MODEL/Measurements'
  Phase6Metadata.protection = 'PHASE6_ASHUGANJ_CCPP_DYNAMIC_MODEL/Protection'
  Phase6Metadata.dc = 'PHASE6_ASHUGANJ_CCPP_DYNAMIC_MODEL/DC Supply'
  Phase6Metadata.breaker = 'PHASE6_ASHUGANJ_CCPP_DYNAMIC_MODEL/Breaker Control'
  Phase6Metadata.machineControl = 'PHASE6_ASHUGANJ_CCPP_DYNAMIC_MODEL/Turbine and AVR'
  Phase6Metadata.results = 'PHASE6_ASHUGANJ_CCPP_DYNAMIC_MODEL/Results'
  Phase6Metadata.sensorNames = {'genInner', 'genTerminal', 'gsutLV', 'gsutHV', 'busIn', 'busOut', 'gatHV', 'lineLocal', 'lineRemote', 'aux', 'grid', 'neutral', 'faultGEN', 'faultLV', 'faultHV', 'faultGIS', 'faultLINE', 'faultGRID', 'faultAUX'}
  Phase6Metadata.summaryNames = {'Generator_P_MW', 'Generator_Q_MVAr', 'Generator_V_kV', 'Generator_I_kA', 'Frequency_Hz', 'Rotor_speed_pu', 'Machine_delta', 'GSUT_HV_I_kA', 'Bus230_V_kV', 'Grid_I_kA', 'Fault_I_kA', 'Relay_pickup', 'Relay_trip', 'GCB_closed', 'Q0_closed', 'Line_local_closed', 'Line_remote_closed', 'DC_V', 'Battery_SOC_pct', 'DC_healthy', 'Auxiliary_V_kV', 'Grid_P_MW', 'Grid_Q_MVAr', 'DC_alarm'}
  R : object (value not decoded)
  S.name = 'normal'
  S.networkProfile = 'PHASE3_BASELINE'
  S.faultEnabled = 0
  S.faultType = '3PH'
  S.faultLocation = 'GIS230'
  S.faultStart_s = 0.15
  S.faultDuration_s = 0.3
  S.stopTime_s = 0.6
  S.faultResistance_ohm = 0.01
  S.groundResistance_ohm = 0.01
  S.protectionEnabled = 1
  S.batteryAvailable = 1
  S.chargerAvailable = 1
  S.dcLossTime_s = Inf
  S.dcRestoreTime_s = Inf
  S.GAT_in = 0
  S.dispatch_MW = 360
  S.relayMask = [1 1 1 1 1 1 1]
  S.breakerFailed = [0 0 0 0 0]
  S.manualOpen = [0 0 0 0 0]
  S.manualOpenTime_s = Inf
  S.generatorTripTime_s = Inf
  S.measurementScale = [1 1 1 1 1 1 1 1 1 1 1 1 1 1 1 1 1 1 1]
values from neighbouring files (symbols this model uses):
  R = struct('out_dir', outDir, 'times_csv', times_csv, 'png', png,      't_op_66_s', t_op_66_s, 't_op_22_s', t_op_22_s, 't_inst_s', t_inst_s,      't_trip_66_s', t_trip_66, 't_trip_22_s', t_trip_22,      'fault_at_s', fault_at_s, 'dt_s', dt,      'Ifault_66_A', Ifault_66_A, 'Ipick_66_A', Ipick_66_A, 'TMS_66', TMS_66,      'Ifault_22_A', Ifault_22_A, 'Ipick_22_A', Ipick_22_A, 'TMS_22', TMS_22,      'sim ...(+220 chars)    [matlab__phase6__run_dynamic_trip_simulation.m]    (also in matlab__tests__test_phase6_dynamic_trip.m = run_dynamic_trip_simulation(out, root); phase6_interactive_settings_before_panel_refresh.m = c.R; realistic_Phase6__scripts__tests__test_phase6_relays.m = phase6_relay_parameters())
  S = struct('out_dir', outDir, 'params_csv', params_csv,      'f_Hz', f_Hz, 'dt_s', dt_s, 'fault_at_s', fault_at_s,      'Iload_66_A', Iload_66_A, 'Ipick_66_A', Ipick_66_A,      'TMS_66', TMS_66, 'Ifault_66_A', Ifault_66_A, 't_op_66_s', t_op_66_s,      'Ipick_22_A', Ipick_22_A, 'TMS_22', TMS_22,      'Ifault_22_A', Ifault_22_A, 't_op_22_s', t_op_22_s,      't_inst_s', t_inst_s, 'pickup_87G_A', 2403.8,  ...(+147 chars)    [matlab__phase6__build_dynamic_protection_sim.m]    (also in matlab__tests__test_phase6_dynamic_trip.m = build_dynamic_protection_sim(out, root); phase6_interactive_settings_before_panel_refresh.m = phase6_normalize_scenario(c.P,S))
undefined symbols (not defined in the file or in its folder): D1, Delta
libraries: spsThreePhaseVIMeasurementLib x18, spsThreePhaseFaultLib x7, spsThreePhaseBreakerLib x5, spsThreePhaseParallelRLCLoadLib x4, spsThreePhasePISectionLineLib x4, spsThreePhaseTransformerTwoWindingsLib x3, spsGroundLib x3, spsSeriesRLCBranchLib x3, spsGroundingTransformerLib x1, spsCurrentMeasurementLib x1, spsSynchronousMachinepuStandardLib x1, spsThreePhaseMutualInductanceZ1Z0Lib x1
(part 1 of 2)
settings Model: Creator=sindi  LastModifiedBy=sindi
settings DataIOCC: SaveOutput=off

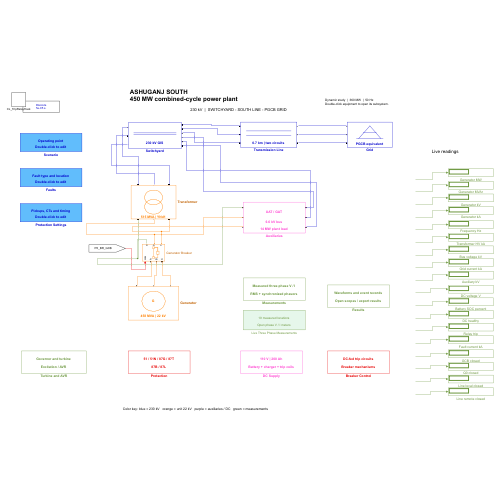
[thumbnail: Simulink's stored preview of the top-level diagram]
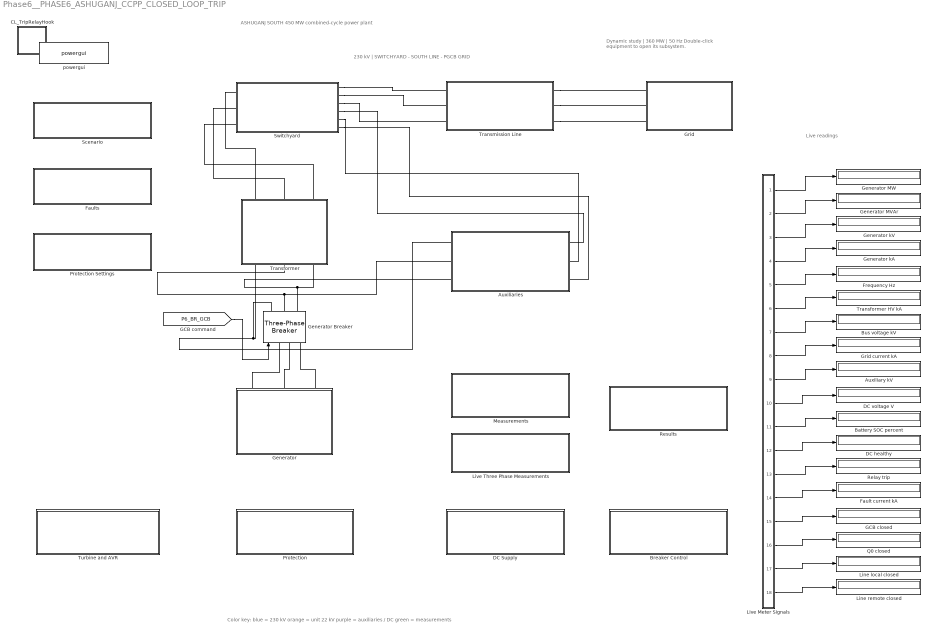
== system Phase6__PHASE6_ASHUGANJ_CCPP_CLOSED_LOOP_TRIP ==
  note: ASHUGANJ SOUTH
      | 450 MW combined-cycle power plant
  note: Dynamic study  |  360 MW  |  50 Hz
      | Double-click equipment to open its subsystem.
  note: 230 kV | SWITCHYARD - SOUTH LINE - PGCB GRID
  note: Live readings
  note: Color key: blue = 230 kV orange = unit 22 kV purple = auxiliaries / DC green = measurements
  Auxiliaries : Subsystem
      mask Display: text(.5,.68,'UAT / GAT','horizontalAlignment','center');text(.5,.38,'6.6 kV bus','horizontalAlignment','center');text(.5,.12,'14 MW plant load','horizontalAlignment','center');
  Auxiliary kV : Display
  Battery SOC percent : Display
  Breaker Control : Subsystem
      mask Display: text(.5,.67,'DC-fed trip circuits','horizontalAlignment','center');text(.5,.30,'Breaker mechanisms','horizontalAlignment','center');
  Bus voltage kV : Display
  CL_TripRelayHook : Subsystem  Description=Task-8 closed-loop trip hook. Intended wiring: DFT/True-RMS measurement @50Hz; IEC SI integrator int(dt/t_op)>=1 to TRIP; ZOH to breaker external control. Placeholder, unconnected; full SPS port mapping pending.
  DC Supply : Subsystem
      mask Display: text(.5,.67,'110 V | 200 Ah','horizontalAlignment','center');text(.5,.30,'Battery + charger + trip coils','horizontalAlignment','center');
  DC healthy : Display
  DC voltage V : Display
  Fault current kA : Display
  Faults : Subsystem
      settings: OpenFcn=phase6_interactive_settings(bdroot);
      mask Display: text(0.5,0.62,'Fault type and location','horizontalAlignment','center');text(0.5,0.25,'Double-click to edit','horizontalAlignment','center');
  Frequency Hz : Display
  GCB closed : Display
  Generator : Subsystem
      mask Display: t=linspace(0,2*pi,80);plot(.5+.23*cos(t),.56+.30*sin(t));text(.5,.58,'G','horizontalAlignment','center');text(.5,.12,'458 MVA | 22 kV','horizontalAlignment','center');
  Generator Breaker : spsThreePhaseBreakerLib/Three-Phase Breaker  InitialState=closed  SwitchA=on  SwitchB=on  SwitchC=on  SwitchTimes="[1/60  5/60]"  External=on  BreakerResistance=0.0001  SnubberResistance=1000000  SnubberCapacitance=inf  Measurements=None
  Generator MVAr : Display
  Generator MW : Display
  Generator kA : Display
  Generator kV : Display
  Grid : Subsystem
      mask Display: plot([.25 .5 .75],[.35 .85 .35]);plot([.35 .65],[.60 .60]);plot([.2 .8],[.35 .35]);text(.5,.13,'PGCB equivalent','horizontalAlignment','center');
  Grid current kA : Display
  Line local closed : Display
  Line remote closed : Display
  Live Meter Signals : Subsystem
  Live Three Phase Measurements : Subsystem
      settings: OpenFcn=open_system([bdroot '/Measurements/Live RMS Readings']);set_param([bdroot '/Measurements/Live RMS Readings'],'ZoomFactor','FitSystem');
      mask Display: text(.5,.65,'19 measured locations','horizontalAlignment','center');text(.5,.27,'Open phase V / I meters','horizontalAlignment','center');
  Measurements : Subsystem
      mask Display: text(.5,.67,'Measured three-phase V / I','horizontalAlignment','center');text(.5,.30,'RMS + synchronized phasors','horizontalAlignment','center');
  Protection : Subsystem
      mask Display: text(.5,.67,'51 / 51N / 87G / 87T','horizontalAlignment','center');text(.5,.30,'87B / 87L','horizontalAlignment','center');
  Protection Settings : Subsystem
      settings: OpenFcn=phase6_interactive_settings(bdroot);
      mask Display: text(0.5,0.62,'Pickups, CTs and timing','horizontalAlignment','center');text(0.5,0.25,'Double-click to edit','horizontalAlignment','center');
  Q0 closed : Display
  Relay trip : Display
  Results : Subsystem
      mask Display: text(.5,.67,'Waveforms and event records','horizontalAlignment','center');text(.5,.30,'Open scopes / export results','horizontalAlignment','center');
  Scenario : Subsystem
      settings: OpenFcn=phase6_interactive_settings(bdroot);
      mask Display: text(0.5,0.62,'Operating point','horizontalAlignment','center');text(0.5,0.25,'Double-click to edit','horizontalAlignment','center');
  Switchyard : Subsystem
      mask Display: plot([.1 .9],[.6 .6]);plot([.1 .9],[.54 .54]);text(.5,.22,'230 kV GIS','horizontalAlignment','center');
  Transformer : Subsystem
      mask Display: t=linspace(0,2*pi,80);plot(.5+.20*cos(t),.64+.22*sin(t));plot(.5+.20*cos(t),.36+.22*sin(t));text(.5,.06,'515 MVA | YNd1','horizontalAlignment','center');
  Transformer HV kA : Display
  Transmission Line : Subsystem
      mask Display: plot([.1 .9],[.65 .65]);plot([.1 .9],[.48 .48]);text(.5,.18,'0.7 km | two circuits','horizontalAlignment','center');
  Turbine and AVR : Subsystem
      mask Display: text(.5,.67,'Governor and turbine','horizontalAlignment','center');text(.5,.30,'Excitation / AVR','horizontalAlignment','center');
  powergui : spspowerguiLib/powergui  Priority=1  SimulationMode=Discrete  SampleTime=5e-05  frequency=50  Iterations=50  frequencyindice=50  Pbase=100e6  ErrMax=1e-7  UnitsV=kV  UnitsW=MW  buscounter=0  FunctionMessages=off  echomessages=off  EnableUseOfTLC=off  CurrentSourceSwitches=off  DisableSnubberDevices=off  DisableRonSwitches=off  DisableVfSwitches=off  DisplayEquations=off  AutomaticDiscreteSolvers=off  SolverType=Tustin/Backward Euler (TBE)  Interpol=off  ExternalGateDelay=off  methode=off  Ts=100  x0status=blocks  SPID=on  SwTol=0  HookPort=off  NonlinearTolerance=1e-4  nMaxIteration=100  ContinueOnMaxIteration=off  RestoreLinks=warning  ResistiveCurrentMeasurement=off  Frange=[0:2:500]  Ylog=off  Xlog=on  ShowGrid=off  save=off  variable=ZData  structure=0  ZoomFFT=off  StartTime=0.0  cycles=1  DisplayStyle=1  fundamental=60  FreqAxis=off  MaxFrequency=1000  frequencyindicesteady=1  RmsSteady=1  display=off
  wires:
  [P6_BR_GCB] -> Generator Breaker/1
  Live Meter Signals/1(Meter 1) -> Generator MW/1
  Live Meter Signals/2(Meter 2) -> Generator MVAr/1
  Live Meter Signals/3(Meter 3) -> Generator kV/1
  Live Meter Signals/4(Meter 4) -> Generator kA/1
  Live Meter Signals/5(Meter 5) -> Frequency Hz/1
  Live Meter Signals/6(Meter 6) -> Transformer HV kA/1
  Live Meter Signals/7(Meter 7) -> Bus voltage kV/1
  Live Meter Signals/8(Meter 8) -> Grid current kA/1
  Live Meter Signals/9(Meter 9) -> Auxiliary kV/1
  Live Meter Signals/10(Meter 10) -> DC voltage V/1
  Live Meter Signals/11(Meter 11) -> Battery SOC percent/1
  Live Meter Signals/12(Meter 12) -> DC healthy/1
  Live Meter Signals/13(Meter 13) -> Relay trip/1
  Live Meter Signals/14(Meter 14) -> Fault current kA/1
  Live Meter Signals/15(Meter 15) -> GCB closed/1
  Live Meter Signals/16(Meter 16) -> Q0 closed/1
  Live Meter Signals/17(Meter 17) -> Line local closed/1
  Live Meter Signals/18(Meter 18) -> Line remote closed/1
  connections:
  Generator/RConn1 -- Generator Breaker/LConn1
  Generator/RConn2 -- Generator Breaker/LConn2
  Generator/RConn3 -- Generator Breaker/LConn3
  Transformer/RConn1 -- Auxiliaries/LConn1 -- Generator Breaker/RConn1
  Generator Breaker/RConn2 -- Transformer/RConn2 -- Auxiliaries/LConn2
  Generator Breaker/RConn3 -- Auxiliaries/LConn3 -- Transformer/RConn3
  Transformer/LConn1 -- Switchyard/LConn1
  Transformer/LConn2 -- Switchyard/LConn2
  Transformer/LConn3 -- Switchyard/LConn3
  Switchyard/RConn1 -- Transmission Line/LConn1
  Switchyard/RConn2 -- Transmission Line/LConn2
  Switchyard/RConn3 -- Transmission Line/LConn3
  Transmission Line/RConn1 -- Grid/LConn1
  Transmission Line/RConn2 -- Grid/LConn2
  Transmission Line/RConn3 -- Grid/LConn3
  Switchyard/RConn4 -- Auxiliaries/RConn1
  Switchyard/RConn5 -- Auxiliaries/RConn2
  Switchyard/RConn6 -- Auxiliaries/RConn3

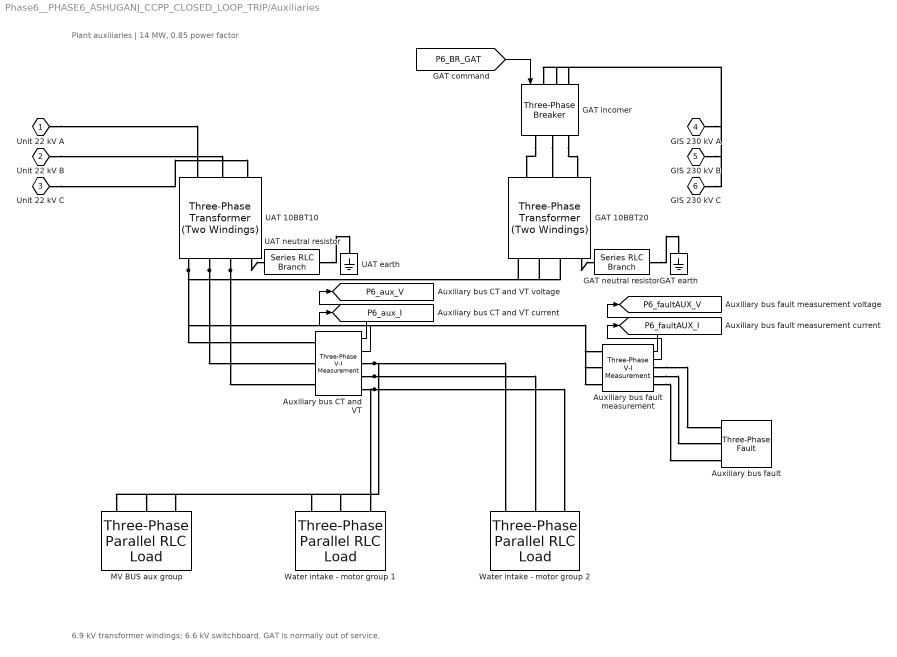
== system Phase6__PHASE6_ASHUGANJ_CCPP_CLOSED_LOOP_TRIP/Auxiliaries ==
  note: Plant auxiliaries | 14 MW, 0.85 power factor
  note: 6.9 kV transformer windings; 6.6 kV switchboard. GAT is normally out of service.
  Auxiliary bus CT and VT : spsThreePhaseVIMeasurementLib/Three-Phase V-I Measurement  VoltageMeasurement=phase-to-ground  SetLabelV=off  LabelV=Vabc  Vpu=off  VpuLL=off  CurrentMeasurement=yes  SetLabelI=off  LabelI=Iabc  Ipu=off  Pbase=100e6  Vbase=500e3  OutputType=Complex  PhasorSimulation=off  PSBequivalent=0
  Auxiliary bus fault : spsThreePhaseFaultLib/Three-Phase Fault  InitialStates=0  FaultA=on  FaultB=on  FaultC=on  GroundFault=off  SwitchTimes=[1000000 1000001]  External=off  SwitchStatus=NaN  FaultResistance=0.01  GroundResistance=0.01  SnubberResistance=1000000000  SnubberCapacitance=inf  Measurements=None
  Auxiliary bus fault measurement : spsThreePhaseVIMeasurementLib/Three-Phase V-I Measurement  VoltageMeasurement=phase-to-ground  SetLabelV=off  LabelV=Vabc  Vpu=off  VpuLL=off  CurrentMeasurement=yes  SetLabelI=off  LabelI=Iabc  Ipu=off  Pbase=100e6  Vbase=500e3  OutputType=Complex  PhasorSimulation=off  PSBequivalent=0
  GAT 10BBT20 : spsThreePhaseTransformerTwoWindingsLib/Three-Phase Transformer (Two Windings)  Winding1Connection=Yg  Winding2Connection=Yn  CoreType=Three single-phase transformers  SetSaturation=off  Hysteresis=off  DataFile='hysteresis'  SetInitialFlux=off  Measurements=None  UNITS=pu  NominalPower=[25000000 50]  Winding1=[230000 0.0025 0.059947894041409]  Winding2=[6900 0.0025 0.059947894041409]  Rm=1086.95652173913  Lm=350.207384175329  L0=0.108  Saturation=[ 0,0 ; 0.0024,1.2 ; 1.0,1.52 ]  InitialFluxes=[ 0.8 , -0.8 , 0.7 ]  BreakLoop=off  DiscreteSolver=Trapezoidal iterative  DataType=off  TransfoNumber=1
  GAT earth : spsGroundLib/Ground  LConnTagsString=a
  GAT incomer : spsThreePhaseBreakerLib/Three-Phase Breaker  InitialState=open  SwitchA=on  SwitchB=on  SwitchC=on  SwitchTimes="[1/60  5/60]"  External=on  BreakerResistance=0.0001  SnubberResistance=1000000  SnubberCapacitance=inf  Measurements=None
  GAT neutral resistor : spsSeriesRLCBranchLib/Series RLC Branch  LConnTagsString=__new0  RConnTagsString=__new0  BranchType=R  Resistance=796.743371481684  Inductance=1e-3  SetiL0=off  InitialCurrent=0  Capacitance=1e-6  Setx0=off  InitialVoltage=0  Measurements=None
  MV BUS aux group : spsThreePhaseParallelRLCLoadLib/Three-Phase Parallel RLC Load  LConnTagsString=A|B|C  Configuration=Y (floating)  NominalVoltage=(6600)*1.00083  Vabc=[1e3 1e3 1e3]  Vabcp=[1e3 1e3 1e3]  NominalFrequency=50  UnbalancedPower=off  ActivePower=9017793.59430605  InductivePower=5588726.52495894  CapacitivePower=0  Pabc=[10e3 9e3 11e3]  QLabc=[100 90 110]  QCabc=[100 90 110]  Pabcp=[10e3 9e3 11e3]  QLabcp=[100 90 110]  QCabcp=[100 90 110]  Measurements=None  LoadType=constant PQ
  UAT 10BBT10 : spsThreePhaseTransformerTwoWindingsLib/Three-Phase Transformer (Two Windings)  Winding1Connection=Delta (D1)  Winding2Connection=Yn  CoreType=Three single-phase transformers  SetSaturation=off  Hysteresis=off  DataFile='hysteresis'  SetInitialFlux=off  Measurements=None  UNITS=pu  NominalPower=[25000000 50]  Winding1=[22000 0.002 0.0524618909304649]  Winding2=[6900 0.002 0.0524618909304649]  Rm=1785.71428571429  Lm=339.297053228746  L0=0.093  Saturation=[ 0,0 ; 0.0024,1.2 ; 1.0,1.52 ]  InitialFluxes=[ 0.8 , -0.8 , 0.7 ]  BreakLoop=off  DiscreteSolver=Trapezoidal iterative  DataType=off  TransfoNumber=1
  UAT earth : spsGroundLib/Ground  LConnTagsString=a
  UAT neutral resistor : spsSeriesRLCBranchLib/Series RLC Branch  LConnTagsString=__new0  RConnTagsString=__new0  BranchType=R  Resistance=796.743371481684  Inductance=1e-3  SetiL0=off  InitialCurrent=0  Capacitance=1e-6  Setx0=off  InitialVoltage=0  Measurements=None
  Water intake - motor group 1 : spsThreePhaseParallelRLCLoadLib/Three-Phase Parallel RLC Load  LConnTagsString=A|B|C  Configuration=Y (floating)  NominalVoltage=(6600)*1.00083  Vabc=[1e3 1e3 1e3]  Vabcp=[1e3 1e3 1e3]  NominalFrequency=50  UnbalancedPower=off  ActivePower=2491103.20284698  InductivePower=1543847.10634225  CapacitivePower=0  Pabc=[10e3 9e3 11e3]  QLabc=[100 90 110]  QCabc=[100 90 110]  Pabcp=[10e3 9e3 11e3]  QLabcp=[100 90 110]  QCabcp=[100 90 110]  Measurements=None  LoadType=constant PQ
  Water intake - motor group 2 : spsThreePhaseParallelRLCLoadLib/Three-Phase Parallel RLC Load  LConnTagsString=A|B|C  Configuration=Y (floating)  NominalVoltage=(6600)*1.00083  Vabc=[1e3 1e3 1e3]  Vabcp=[1e3 1e3 1e3]  NominalFrequency=50  UnbalancedPower=off  ActivePower=2491103.20284698  InductivePower=1543847.10634225  CapacitivePower=0  Pabc=[10e3 9e3 11e3]  QLabc=[100 90 110]  QCabc=[100 90 110]  Pabcp=[10e3 9e3 11e3]  QLabcp=[100 90 110]  QCabcp=[100 90 110]  Measurements=None  LoadType=constant PQ
  Unit 22 kV A : PMIOPort  Side=Left
  Unit 22 kV B : PMIOPort  Port=2  Side=Left
  Unit 22 kV C : PMIOPort  Port=3  Side=Left
  GIS 230 kV A : PMIOPort  Port=4  Side=Right
  GIS 230 kV B : PMIOPort  Port=5  Side=Right
  GIS 230 kV C : PMIOPort  Port=6  Side=Right
  tag scope: P6_aux_I=global, P6_aux_V=global, P6_faultAUX_I=global, P6_faultAUX_V=global
  wires:
  [P6_BR_GAT] -> GAT incomer/1
  Auxiliary bus CT and VT/1 -> [P6_aux_V]
  Auxiliary bus CT and VT/2 -> [P6_aux_I]
  Auxiliary bus fault measurement/1 -> [P6_faultAUX_V]
  Auxiliary bus fault measurement/2 -> [P6_faultAUX_I]
  connections:
  UAT 10BBT10/RConn4 -- UAT neutral resistor/LConn1
  UAT neutral resistor/RConn1 -- UAT earth/LConn1
  GAT 10BBT20/RConn4 -- GAT neutral resistor/LConn1
  GAT neutral resistor/RConn1 -- GAT earth/LConn1
  Unit 22 kV A/RConn1 -- UAT 10BBT10/LConn1
  Unit 22 kV B/RConn1 -- UAT 10BBT10/LConn2
  Unit 22 kV C/RConn1 -- UAT 10BBT10/LConn3
  GIS 230 kV A/RConn1 -- GAT incomer/LConn1
  GIS 230 kV B/RConn1 -- GAT incomer/LConn2
  GIS 230 kV C/RConn1 -- GAT incomer/LConn3
  GAT incomer/RConn1 -- GAT 10BBT20/LConn1
  GAT incomer/RConn2 -- GAT 10BBT20/LConn2
  GAT incomer/RConn3 -- GAT 10BBT20/LConn3
  GAT 10BBT20/RConn1 -- UAT 10BBT10/RConn1 -- Auxiliary bus CT and VT/LConn1 -- Auxiliary bus fault measurement/LConn1
  GAT 10BBT20/RConn2 -- UAT 10BBT10/RConn2 -- Auxiliary bus CT and VT/LConn2 -- Auxiliary bus fault measurement/LConn2
  GAT 10BBT20/RConn3 -- UAT 10BBT10/RConn3 -- Auxiliary bus CT and VT/LConn3 -- Auxiliary bus fault measurement/LConn3
  MV BUS aux group/LConn1 -- Auxiliary bus CT and VT/RConn1 -- Water intake - motor group 1/LConn1 -- Water intake - motor group 2/LConn1
  MV BUS aux group/LConn2 -- Auxiliary bus CT and VT/RConn2 -- Water intake - motor group 1/LConn2 -- Water intake - motor group 2/LConn2
  MV BUS aux group/LConn3 -- Auxiliary bus CT and VT/RConn3 -- Water intake - motor group 1/LConn3 -- Water intake - motor group 2/LConn3
  Auxiliary bus fault measurement/RConn1 -- Auxiliary bus fault/LConn1
  Auxiliary bus fault measurement/RConn2 -- Auxiliary bus fault/LConn2
  Auxiliary bus fault measurement/RConn3 -- Auxiliary bus fault/LConn3

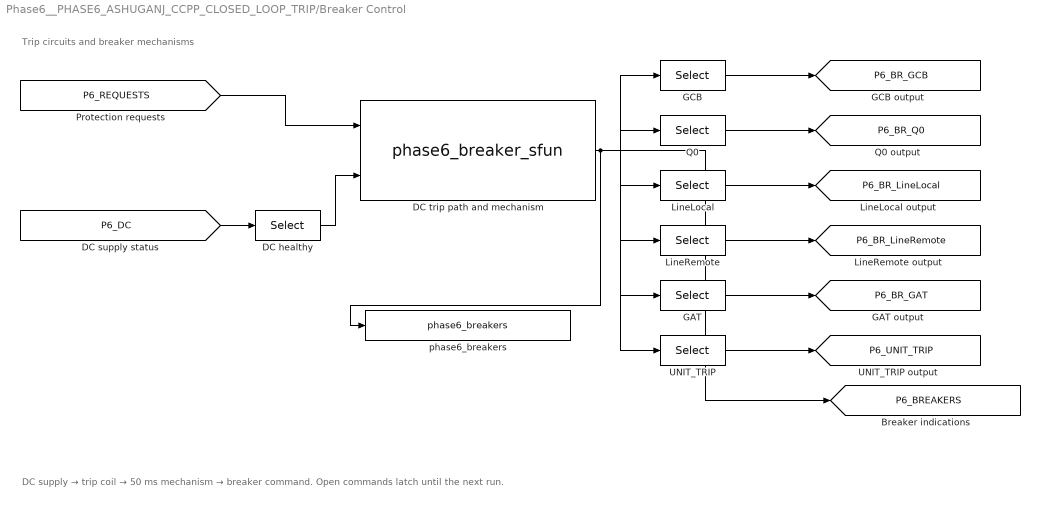
== system Phase6__PHASE6_ASHUGANJ_CCPP_CLOSED_LOOP_TRIP/Breaker Control ==
  note: Trip circuits and breaker mechanisms
  note: DC supply → trip coil → 50 ms mechanism → breaker command. Open commands latch until the next run.
  DC healthy : Selector  IndexOptions=Index vector (dialog)  Indices=6  OutputSizes=1
  DC trip path and mechanism : M-S-Function  FunctionName=phase6_breaker_sfun  Parameters=C,S
  GAT : Selector  IndexOptions=Index vector (dialog)  Indices=5  OutputSizes=1
  GCB : Selector  IndexOptions=Index vector (dialog)  Indices=1  OutputSizes=1
  LineLocal : Selector  IndexOptions=Index vector (dialog)  Indices=3  OutputSizes=1
  LineRemote : Selector  IndexOptions=Index vector (dialog)  Indices=4  OutputSizes=1
  Q0 : Selector  IndexOptions=Index vector (dialog)  Indices=2  OutputSizes=1
  UNIT_TRIP : Selector  IndexOptions=Index vector (dialog)  Indices=6  OutputSizes=1
  phase6_breakers : ToWorkspace  VariableName=phase6_breakers  SaveFormat=Timeseries  SampleTime=-1
  tag scope: P6_BREAKERS=global, P6_BR_GAT=global, P6_BR_GCB=global, P6_BR_LineLocal=global, P6_BR_LineRemote=global, P6_BR_Q0=global, P6_UNIT_TRIP=global
  wires:
  [P6_REQUESTS] -> DC trip path and mechanism/1
  [P6_DC] -> DC healthy/1
  DC healthy/1 -> DC trip path and mechanism/2
  DC trip path and mechanism/1 -> [P6_BREAKERS], GCB/1, Q0/1, LineLocal/1, LineRemote/1, GAT/1, UNIT_TRIP/1, phase6_breakers/1
  GCB/1 -> [P6_BR_GCB]
  Q0/1 -> [P6_BR_Q0]
  LineLocal/1 -> [P6_BR_LineLocal]
  LineRemote/1 -> [P6_BR_LineRemote]
  GAT/1 -> [P6_BR_GAT]
  UNIT_TRIP/1 -> [P6_UNIT_TRIP]

== system Phase6__PHASE6_ASHUGANJ_CCPP_CLOSED_LOOP_TRIP/CL_TripRelayHook ==
  SI_integrator : Gain
  TRIP_out : Terminator
  inv_top : Constant
  wires:
  inv_top/1 -> SI_integrator/1
  SI_integrator/1 -> TRIP_out/1

== system Phase6__PHASE6_ASHUGANJ_CCPP_CLOSED_LOOP_TRIP/DC Supply ==
  note: 110 V station DC supply
  note: AC supply → charger | battery ↔ DC bus → control loads and trip coils
  note: 55-cell, 200 Ah study bank. The bus solves battery resistance, charger limits, load demand and SOC at each time step.
  AC supply magnitude : Fcn  Expr=sqrt((u(1)^2+u(2)^2+u(3)^2)/3)*sqrt(3)/6600
  Auxiliary phase voltage : Selector  IndexOptions=Index vector (dialog)  Indices=[55 56 57]  OutputSizes=1
  Battery charger and DC bus : M-S-Function  FunctionName=phase6_dc_sfun  Parameters=D,S
  DC voltage current and SOC : Scope
  Trip coil demand : Fcn  Expr=u(1)+u(2)+u(3)+u(4)+u(5)+u(6)>0
  phase6_dc : ToWorkspace  VariableName=phase6_dc  SaveFormat=Timeseries  SampleTime=-1
  tag scope: P6_DC=global
  wires:
  [P6_RMS] -> Auxiliary phase voltage/1
  Auxiliary phase voltage/1 -> AC supply magnitude/1
  AC supply magnitude/1 -> Battery charger and DC bus/1
  [P6_REQUESTS] -> Trip coil demand/1
  Trip coil demand/1 -> Battery charger and DC bus/2
  Battery charger and DC bus/1 -> [P6_DC], phase6_dc/1, DC voltage current and SOC/1

== system Phase6__PHASE6_ASHUGANJ_CCPP_CLOSED_LOOP_TRIP/Faults ==

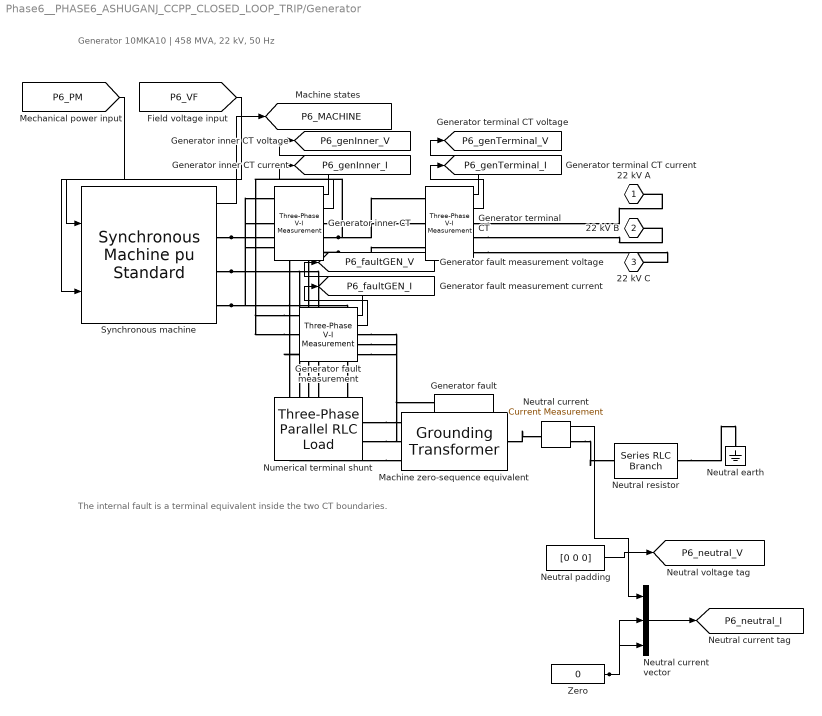
== system Phase6__PHASE6_ASHUGANJ_CCPP_CLOSED_LOOP_TRIP/Generator ==
  note: Generator 10MKA10 | 458 MVA, 22 kV, 50 Hz
  note: The internal fault is a terminal equivalent inside the two CT boundaries.
  Generator fault : spsThreePhaseFaultLib/Three-Phase Fault  InitialStates=0  FaultA=on  FaultB=on  FaultC=on  GroundFault=off  SwitchTimes=[1000000 1000001]  External=off  SwitchStatus=NaN  FaultResistance=0.01  GroundResistance=0.01  SnubberResistance=1000000000  SnubberCapacitance=inf  Measurements=None
  Generator fault measurement : spsThreePhaseVIMeasurementLib/Three-Phase V-I Measurement  VoltageMeasurement=phase-to-ground  SetLabelV=off  LabelV=Vabc  Vpu=off  VpuLL=off  CurrentMeasurement=yes  SetLabelI=off  LabelI=Iabc  Ipu=off  Pbase=100e6  Vbase=500e3  OutputType=Complex  PhasorSimulation=off  PSBequivalent=0
  Generator inner CT : spsThreePhaseVIMeasurementLib/Three-Phase V-I Measurement  VoltageMeasurement=phase-to-ground  SetLabelV=off  LabelV=Vabc  Vpu=off  VpuLL=off  CurrentMeasurement=yes  SetLabelI=off  LabelI=Iabc  Ipu=off  Pbase=100e6  Vbase=500e3  OutputType=Complex  PhasorSimulation=off  PSBequivalent=0
  Generator terminal CT : spsThreePhaseVIMeasurementLib/Three-Phase V-I Measurement  VoltageMeasurement=phase-to-ground  SetLabelV=off  LabelV=Vabc  Vpu=off  VpuLL=off  CurrentMeasurement=yes  SetLabelI=off  LabelI=Iabc  Ipu=off  Pbase=100e6  Vbase=500e3  OutputType=Complex  PhasorSimulation=off  PSBequivalent=0
  Machine zero-sequence equivalent : spsGroundingTransformerLib/Grounding Transformer   UNITS=pu  NominalPower=[458000000 50]  NominalVoltage=22000  ZeroSequenceImpedance_pu=[0.00126328512396694 0.128]  MagnetizationBranch_pu=[10000000 10000000]  ZeroSequenceImpedance_SI=[0.052083 589.05]  MagnetizationBranch_SI=[1041.7 3.927e+005]  Measurements=None
  Neutral current : spsCurrentMeasurementLib/Current Measurement  PhasorSimulation=off  OutputType=Complex  PSBequivalent=0
  Neutral current vector : Mux  Inputs=3
  Neutral earth : spsGroundLib/Ground  LConnTagsString=a
  Neutral padding : Constant  Value=[0 0 0]
  Neutral resistor : spsSeriesRLCBranchLib/Series RLC Branch  LConnTagsString=__new0  RConnTagsString=__new0  BranchType=R  Resistance=1750.77333333333  Inductance=1e-3  SetiL0=off  InitialCurrent=0  Capacitance=1e-6  Setx0=off  InitialVoltage=0  Measurements=None
  Numerical terminal shunt : spsThreePhaseParallelRLCLoadLib/Three-Phase Parallel RLC Load  LConnTagsString=A|B|C  Configuration=Y (grounded)  NominalVoltage=22000  Vabc=[1e3 1e3 1e3]  Vabcp=[1e3 1e3 1e3]  NominalFrequency=50  UnbalancedPower=off  ActivePower=10  InductivePower=0  CapacitivePower=0  Pabc=[10e3 9e3 11e3]  QLabc=[100 90 110]  QCabc=[100 90 110]  Pabcp=[10e3 9e3 11e3]  QLabcp=[100 90 110]  QCabcp=[100 90 110]  Measurements=None  LoadType=constant Z
  Synchronous machine : spsSynchronousMachinepuStandardLib/Synchronous Machine pu Standard  PresetModel=No  MechanicalLoad=Mechanical power Pm  ShowDetailedParameters=on  RotorType=Round  Units=per unit standard parameters  MeasurementBus=on  NominalParameters=[458000000 22000 50]  Reactances1=[1.783 0.3256 0.2608 1.751 0.5087 0.2593 0.2027]  Reactances2=[2.24 0.17 0.12 1.02 0.13 0.08]  dAxisTimeConstants=Open-circuit  qAxisTimeConstants=Open-circuit  TimeConstants1="[ 4.4849  0.0681  0.1  ]"  TimeConstants2=[7.547 0.045 0.839 0.07]  TimeConstants3="[  4.49  0.0681  0.0513  ]"  TimeConstants4=[ 8.0, 0.03, 0.3371, 0.0295 ]  TimeConstants5=[ 1.01, 0.053, 0.1 ]  TimeConstants6=[ 1.3201, 0.023, 1.0, 0.07 ]  TimeConstants7=[0.012 0.003 0.003]  TimeConstants8=[ 1.3201, 0.0231, 0.3371, 0.0295 ]  StatorResistance=0.000842190082644628  Mechanical=[5.287 0 1]  PolePairs=20  InitialConditions=[0 -61.5749 0.788336 0.788336 0.788336 -27.1695 -147.17 92.8305 1.78658]  SetSaturation=off  Saturation=[0.6404,0.7127,0.8441,0.9214,0.9956,1.082,1.19,1.316,1.457;0.7,0.7698,0.8872,0.9466,0.9969,1.046,1.1,1.151,1.201]  LoadFlowParameters=[1,0,0,0,0]  TsPowergui=0  TsBlock=-1  IterativeModel=Trapezoidal non iterative  IterativeDiscreteModel=Trapezoidal robust  BusType=PV  Pref=360000000  Qref=0  Qmin=-inf  Qmax=inf  PLF=0  QLF=0
  Zero : Constant  Value=0
  22 kV A : PMIOPort  Side=Right
  22 kV B : PMIOPort  Port=2  Side=Right
  22 kV C : PMIOPort  Port=3  Side=Right
  tag scope: P6_MACHINE=global, P6_faultGEN_I=global, P6_faultGEN_V=global, P6_genInner_I=global, P6_genInner_V=global, P6_genTerminal_I=global, P6_genTerminal_V=global, P6_neutral_I=global, P6_neutral_V=global
  wires:
  Neutral padding/1 -> [P6_neutral_V]
  Neutral current/1 -> Neutral current vector/1
  Zero/1 -> Neutral current vector/2, Neutral current vector/3
  Neutral current vector/1 -> [P6_neutral_I]
  Generator inner CT/1 -> [P6_genInner_V]
  Generator inner CT/2 -> [P6_genInner_I]
  Generator fault measurement/1 -> [P6_faultGEN_V]
  Generator fault measurement/2 -> [P6_faultGEN_I]
  Generator terminal CT/1 -> [P6_genTerminal_V]
  Generator terminal CT/2 -> [P6_genTerminal_I]
  Synchronous machine/1 -> [P6_MACHINE]
  [P6_PM] -> Synchronous machine/1
  [P6_VF] -> Synchronous machine/2
  connections:
  Machine zero-sequence equivalent/LConn1 -- Synchronous machine/RConn1 -- Numerical terminal shunt/LConn1 -- Generator inner CT/LConn1
  Machine zero-sequence equivalent/LConn2 -- Synchronous machine/RConn2 -- Numerical terminal shunt/LConn2 -- Generator inner CT/LConn2
  Machine zero-sequence equivalent/LConn3 -- Synchronous machine/RConn3 -- Numerical terminal shunt/LConn3 -- Generator inner CT/LConn3
  Machine zero-sequence equivalent/RConn1 -- Neutral current/LConn1
  Neutral current/RConn1 -- Neutral resistor/LConn1
  Neutral resistor/RConn1 -- Neutral earth/LConn1
  Generator fault measurement/LConn1 -- Generator inner CT/RConn1 -- Generator terminal CT/LConn1
  Generator fault measurement/LConn2 -- Generator inner CT/RConn2 -- Generator terminal CT/LConn2
  Generator fault measurement/LConn3 -- Generator inner CT/RConn3 -- Generator terminal CT/LConn3
  Generator fault measurement/RConn1 -- Generator fault/LConn1
  Generator fault measurement/RConn2 -- Generator fault/LConn2
  Generator fault measurement/RConn3 -- Generator fault/LConn3
  Generator terminal CT/RConn1 -- 22 kV A/RConn1
  Generator terminal CT/RConn2 -- 22 kV B/RConn1
  Generator terminal CT/RConn3 -- 22 kV C/RConn1

== system Phase6__PHASE6_ASHUGANJ_CCPP_CLOSED_LOOP_TRIP/Grid ==
  note: PGCB equivalent | 230 kV, 50 Hz
  note: PHASE3 BASELINE
  Grid CT and VT : spsThreePhaseVIMeasurementLib/Three-Phase V-I Measurement  VoltageMeasurement=phase-to-ground  SetLabelV=off  LabelV=Vabc  Vpu=off  VpuLL=off  CurrentMeasurement=yes  SetLabelI=off  LabelI=Iabc  Ipu=off  Pbase=100e6  Vbase=500e3  OutputType=Complex  PhasorSimulation=off  PSBequivalent=0
  Grid sequence impedance : spsThreePhaseMutualInductanceZ1Z0Lib/Three-Phase Mutual Inductance Z1-Z0  LConnTagsString=a|b|c  RConnTagsString=A|B|C  PositiveSequence=[0 0.00845370972980081]  ZeroSequence=[0 0.0126805645947012]
      settings: AttributesFormatString=\n
  PGCB voltage source : spsThreePhaseSourceLib/Three-Phase Source  InternalConnection=Yg  VoltagePhases=off  Voltage=(230000)*1  PhaseAngle=0  Voltage_phases=[25e3 25e3 25e3]/sqrt(3)  PhaseAngles_phases=[0 -120 +120]  Frequency=50  NonIdealSource=off  SpecifyImpedance=off  Resistance=0.8929  Inductance=16.58e-3  ShortCircuitLevel=100e6  BaseVoltage=230000  XRratio=7  BusType=swing  Pref=10e3  Qref=0  Prefabc=[10e3, 10e3, 10e3]  Qrefabc=[0, 0, 0]  Qmin=-inf  Qmax=inf
  Remote bus fault : spsThreePhaseFaultLib/Three-Phase Fault  InitialStates=0  FaultA=on  FaultB=on  FaultC=on  GroundFault=off  SwitchTimes=[1000000 1000001]  External=off  SwitchStatus=NaN  FaultResistance=0.01  GroundResistance=0.01  SnubberResistance=1000000000  SnubberCapacitance=inf  Measurements=None
  Remote bus fault measurement : spsThreePhaseVIMeasurementLib/Three-Phase V-I Measurement  VoltageMeasurement=phase-to-ground  SetLabelV=off  LabelV=Vabc  Vpu=off  VpuLL=off  CurrentMeasurement=yes  SetLabelI=off  LabelI=Iabc  Ipu=off  Pbase=100e6  Vbase=500e3  OutputType=Complex  PhasorSimulation=off  PSBequivalent=0
  230 kV A : PMIOPort  Side=Left
  230 kV B : PMIOPort  Port=2  Side=Left
  230 kV C : PMIOPort  Port=3  Side=Left
  tag scope: P6_faultGRID_I=global, P6_faultGRID_V=global, P6_grid_I=global, P6_grid_V=global
  wires:
  Grid CT and VT/1 -> [P6_grid_V]
  Grid CT and VT/2 -> [P6_grid_I]
  Remote bus fault measurement/1 -> [P6_faultGRID_V]
  Remote bus fault measurement/2 -> [P6_faultGRID_I]
  connections:
  Grid CT and VT/LConn1 -- 230 kV A/RConn1 -- Remote bus fault measurement/LConn1
  Grid CT and VT/LConn2 -- 230 kV B/RConn1 -- Remote bus fault measurement/LConn2
  Grid CT and VT/LConn3 -- 230 kV C/RConn1 -- Remote bus fault measurement/LConn3
  Grid CT and VT/RConn1 -- Grid sequence impedance/LConn1
  Grid CT and VT/RConn2 -- Grid sequence impedance/LConn2
  Grid CT and VT/RConn3 -- Grid sequence impedance/LConn3
  Grid sequence impedance/RConn1 -- PGCB voltage source/RConn1
  Grid sequence impedance/RConn2 -- PGCB voltage source/RConn2
  Grid sequence impedance/RConn3 -- PGCB voltage source/RConn3
  Remote bus fault measurement/RConn1 -- Remote bus fault/LConn1
  Remote bus fault measurement/RConn2 -- Remote bus fault/LConn2
  Remote bus fault measurement/RConn3 -- Remote bus fault/LConn3

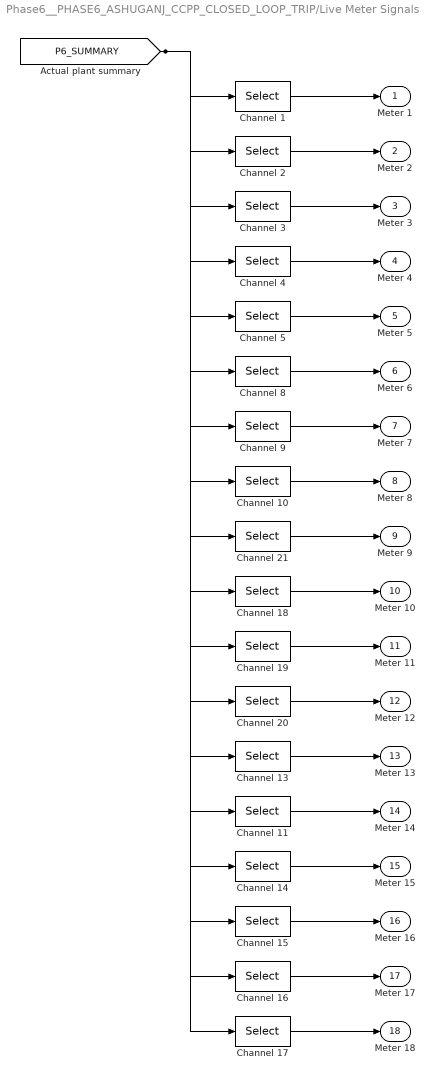
== system Phase6__PHASE6_ASHUGANJ_CCPP_CLOSED_LOOP_TRIP/Live Meter Signals ==
  Channel 1 : Selector  InputPortWidth=24  IndexOptions=Index vector (dialog)  Indices=1  OutputSizes=1
  Channel 10 : Selector  InputPortWidth=24  IndexOptions=Index vector (dialog)  Indices=10  OutputSizes=1
  Channel 11 : Selector  InputPortWidth=24  IndexOptions=Index vector (dialog)  Indices=11  OutputSizes=1
  Channel 13 : Selector  InputPortWidth=24  IndexOptions=Index vector (dialog)  Indices=13  OutputSizes=1
  Channel 14 : Selector  InputPortWidth=24  IndexOptions=Index vector (dialog)  Indices=14  OutputSizes=1
  Channel 15 : Selector  InputPortWidth=24  IndexOptions=Index vector (dialog)  Indices=15  OutputSizes=1
  Channel 16 : Selector  InputPortWidth=24  IndexOptions=Index vector (dialog)  Indices=16  OutputSizes=1
  Channel 17 : Selector  InputPortWidth=24  IndexOptions=Index vector (dialog)  Indices=17  OutputSizes=1
  Channel 18 : Selector  InputPortWidth=24  IndexOptions=Index vector (dialog)  Indices=18  OutputSizes=1
  Channel 19 : Selector  InputPortWidth=24  IndexOptions=Index vector (dialog)  Indices=19  OutputSizes=1
  Channel 2 : Selector  InputPortWidth=24  IndexOptions=Index vector (dialog)  Indices=2  OutputSizes=1
  Channel 20 : Selector  InputPortWidth=24  IndexOptions=Index vector (dialog)  Indices=20  OutputSizes=1
  Channel 21 : Selector  InputPortWidth=24  IndexOptions=Index vector (dialog)  Indices=21  OutputSizes=1
  Channel 3 : Selector  InputPortWidth=24  IndexOptions=Index vector (dialog)  Indices=3  OutputSizes=1
  Channel 4 : Selector  InputPortWidth=24  IndexOptions=Index vector (dialog)  Indices=4  OutputSizes=1
  Channel 5 : Selector  InputPortWidth=24  IndexOptions=Index vector (dialog)  Indices=5  OutputSizes=1
  Channel 8 : Selector  InputPortWidth=24  IndexOptions=Index vector (dialog)  Indices=8  OutputSizes=1
  Channel 9 : Selector  InputPortWidth=24  IndexOptions=Index vector (dialog)  Indices=9  OutputSizes=1
  Meter 1 : Outport
  Meter 2 : Outport  Port=2
  Meter 3 : Outport  Port=3
  Meter 4 : Outport  Port=4
  Meter 5 : Outport  Port=5
  Meter 6 : Outport  Port=6
  Meter 7 : Outport  Port=7
  Meter 8 : Outport  Port=8
  Meter 9 : Outport  Port=9
  Meter 10 : Outport  Port=10
  Meter 11 : Outport  Port=11
  Meter 12 : Outport  Port=12
  Meter 13 : Outport  Port=13
  Meter 14 : Outport  Port=14
  Meter 15 : Outport  Port=15
  Meter 16 : Outport  Port=16
  Meter 17 : Outport  Port=17
  Meter 18 : Outport  Port=18
  wires:
  [P6_SUMMARY] -> Channel 1/1, Channel 2/1, Channel 3/1, Channel 4/1, Channel 5/1, Channel 8/1, Channel 9/1, Channel 10/1, Channel 21/1, Channel 18/1, Channel 19/1, Channel 20/1, Channel 13/1, Channel 11/1, Channel 14/1, Channel 15/1, Channel 16/1, Channel 17/1
  Channel 1/1 -> Meter 1/1
  Channel 2/1 -> Meter 2/1
  Channel 3/1 -> Meter 3/1
  Channel 4/1 -> Meter 4/1
  Channel 5/1 -> Meter 5/1
  Channel 8/1 -> Meter 6/1
  Channel 9/1 -> Meter 7/1
  Channel 10/1 -> Meter 8/1
  Channel 21/1 -> Meter 9/1
  Channel 18/1 -> Meter 10/1
  Channel 19/1 -> Meter 11/1
  Channel 20/1 -> Meter 12/1
  Channel 13/1 -> Meter 13/1
  Channel 11/1 -> Meter 14/1
  Channel 14/1 -> Meter 15/1
  Channel 15/1 -> Meter 16/1
  Channel 16/1 -> Meter 17/1
  Channel 17/1 -> Meter 18/1

== system Phase6__PHASE6_ASHUGANJ_CCPP_CLOSED_LOOP_TRIP/Live Three Phase Measurements ==

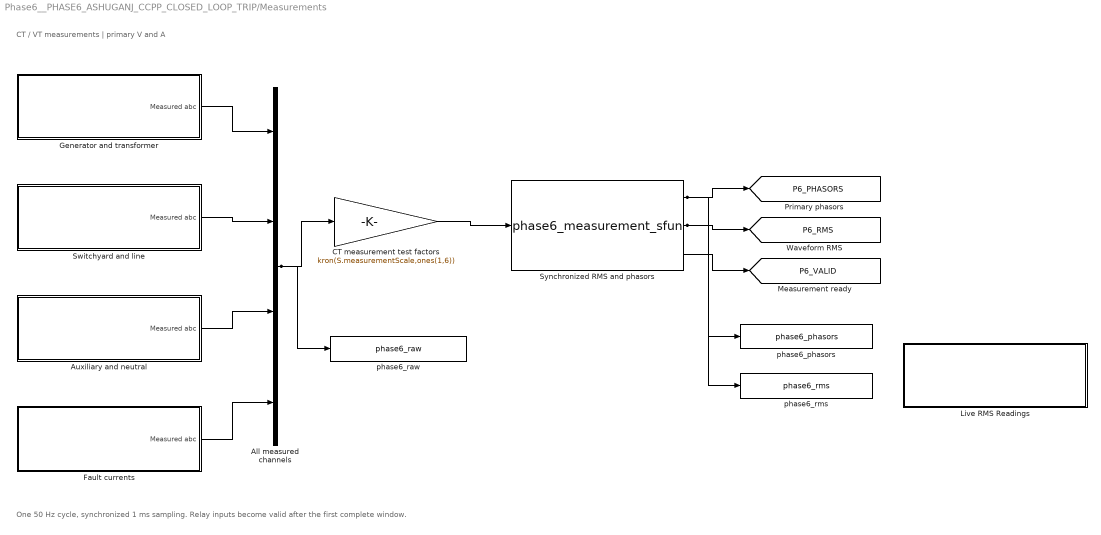
== system Phase6__PHASE6_ASHUGANJ_CCPP_CLOSED_LOOP_TRIP/Measurements ==
  note: CT / VT measurements | primary V and A
  note: One 50 Hz cycle, synchronized 1 ms sampling. Relay inputs become valid after the first complete window.
  All measured channels : Mux
  Auxiliary and neutral : Subsystem
  CT measurement test factors : Gain  Gain=kron(S.measurementScale,ones(1,6))
  Fault currents : Subsystem
  Generator and transformer : Subsystem
  Live RMS Readings : Subsystem
  Switchyard and line : Subsystem
  Synchronized RMS and phasors : M-S-Function  FunctionName=phase6_measurement_sfun
  phase6_phasors : ToWorkspace  VariableName=phase6_phasors  SaveFormat=Timeseries  SampleTime=-1
  phase6_raw : ToWorkspace  VariableName=phase6_raw  SaveFormat=Timeseries  SampleTime=0.0002
  phase6_rms : ToWorkspace  VariableName=phase6_rms  SaveFormat=Timeseries  SampleTime=-1
  tag scope: P6_PHASORS=global, P6_RMS=global, P6_VALID=global
  wires:
  Generator and transformer/1(Measured abc) -> All measured channels/1
  Switchyard and line/1(Measured abc) -> All measured channels/2
  Auxiliary and neutral/1(Measured abc) -> All measured channels/3
  Fault currents/1(Measured abc) -> All measured channels/4
  All measured channels/1 -> CT measurement test factors/1, phase6_raw/1
  CT measurement test factors/1 -> Synchronized RMS and phasors/1
  Synchronized RMS and phasors/1 -> [P6_PHASORS], phase6_phasors/1
  Synchronized RMS and phasors/2 -> [P6_RMS], phase6_rms/1
  Synchronized RMS and phasors/3 -> [P6_VALID]

== system Phase6__PHASE6_ASHUGANJ_CCPP_CLOSED_LOOP_TRIP/Protection ==
  note: 51 / 51N 87G 87T 87B 87L
  note: Measured currents → CT ratios → pickup / timing → trip request
  note: Open the algorithm block to inspect the tested equations. Trip requests pass through the DC supply and breaker mechanism.
  Pickup and relay timing : M-S-Function  FunctionName=phase6_relay_sfun  Parameters=R,S
  Relay pickup and timing : Scope
  phase6_relay : ToWorkspace  VariableName=phase6_relay  SaveFormat=Timeseries  SampleTime=-1
  tag scope: P6_RELAY=global, P6_REQUESTS=global
  wires:
  [P6_PHASORS] -> Pickup and relay timing/1
  [P6_VALID] -> Pickup and relay timing/2
  Pickup and relay timing/1 -> [P6_RELAY], phase6_relay/1, Relay pickup and timing/1
  Pickup and relay timing/2 -> [P6_REQUESTS]

== system Phase6__PHASE6_ASHUGANJ_CCPP_CLOSED_LOOP_TRIP/Protection Settings ==

== system Phase6__PHASE6_ASHUGANJ_CCPP_CLOSED_LOOP_TRIP/Results ==
  note: Dynamic measurements and event records
  note: All records come from this simulation. Run export_phase6_results to create labelled plots and CSV tables.
  Dynamic response : Scope
  Plant quantities : M-S-Function  FunctionName=phase6_monitor_sfun
  phase6_summary : ToWorkspace  VariableName=phase6_summary  SaveFormat=Timeseries  SampleTime=-1
  tag scope: P6_SUMMARY=global
  wires:
  [P6_PHASORS] -> Plant quantities/1
  [P6_MACHINE_RECORD] -> Plant quantities/2
  [P6_RELAY] -> Plant quantities/3
  [P6_BREAKERS] -> Plant quantities/4
  [P6_DC] -> Plant quantities/5
  Plant quantities/1 -> [P6_SUMMARY], phase6_summary/1, Dynamic response/1

== system Phase6__PHASE6_ASHUGANJ_CCPP_CLOSED_LOOP_TRIP/Scenario ==

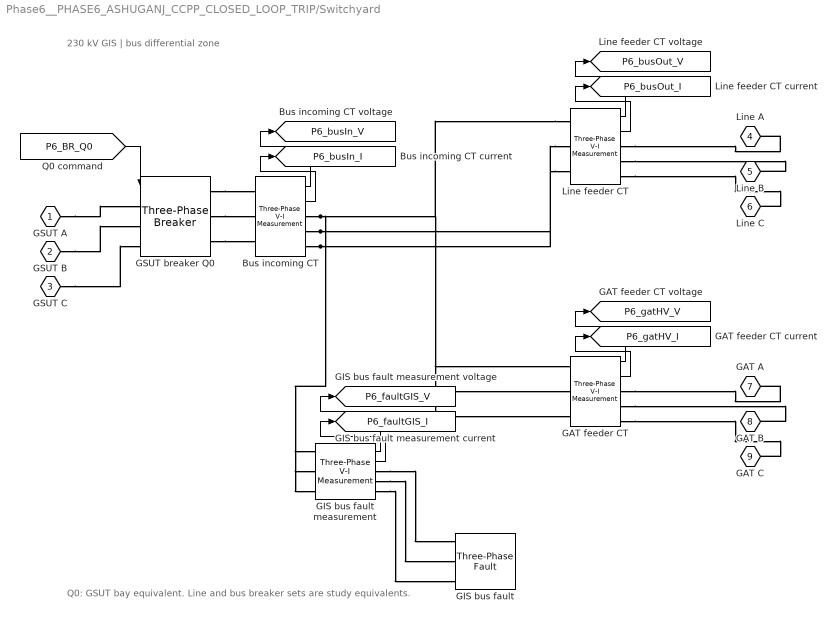
== system Phase6__PHASE6_ASHUGANJ_CCPP_CLOSED_LOOP_TRIP/Switchyard ==
  note: 230 kV GIS | bus differential zone
  note: Q0: GSUT bay equivalent. Line and bus breaker sets are study equivalents.
  Bus incoming CT : spsThreePhaseVIMeasurementLib/Three-Phase V-I Measurement  VoltageMeasurement=phase-to-ground  SetLabelV=off  LabelV=Vabc  Vpu=off  VpuLL=off  CurrentMeasurement=yes  SetLabelI=off  LabelI=Iabc  Ipu=off  Pbase=100e6  Vbase=500e3  OutputType=Complex  PhasorSimulation=off  PSBequivalent=0
  GAT feeder CT : spsThreePhaseVIMeasurementLib/Three-Phase V-I Measurement  VoltageMeasurement=phase-to-ground  SetLabelV=off  LabelV=Vabc  Vpu=off  VpuLL=off  CurrentMeasurement=yes  SetLabelI=off  LabelI=Iabc  Ipu=off  Pbase=100e6  Vbase=500e3  OutputType=Complex  PhasorSimulation=off  PSBequivalent=0
  GIS bus fault : spsThreePhaseFaultLib/Three-Phase Fault  InitialStates=0  FaultA=on  FaultB=on  FaultC=on  GroundFault=off  SwitchTimes=[1000000 1000001]  External=off  SwitchStatus=NaN  FaultResistance=0.01  GroundResistance=0.01  SnubberResistance=1000000000  SnubberCapacitance=inf  Measurements=None
  GIS bus fault measurement : spsThreePhaseVIMeasurementLib/Three-Phase V-I Measurement  VoltageMeasurement=phase-to-ground  SetLabelV=off  LabelV=Vabc  Vpu=off  VpuLL=off  CurrentMeasurement=yes  SetLabelI=off  LabelI=Iabc  Ipu=off  Pbase=100e6  Vbase=500e3  OutputType=Complex  PhasorSimulation=off  PSBequivalent=0
  GSUT breaker Q0 : spsThreePhaseBreakerLib/Three-Phase Breaker  InitialState=closed  SwitchA=on  SwitchB=on  SwitchC=on  SwitchTimes="[1/60  5/60]"  External=on  BreakerResistance=0.0001  SnubberResistance=1000000  SnubberCapacitance=inf  Measurements=None
  Line feeder CT : spsThreePhaseVIMeasurementLib/Three-Phase V-I Measurement  VoltageMeasurement=phase-to-ground  SetLabelV=off  LabelV=Vabc  Vpu=off  VpuLL=off  CurrentMeasurement=yes  SetLabelI=off  LabelI=Iabc  Ipu=off  Pbase=100e6  Vbase=500e3  OutputType=Complex  PhasorSimulation=off  PSBequivalent=0
  GSUT A : PMIOPort  Side=Left
  GSUT B : PMIOPort  Port=2  Side=Left
  GSUT C : PMIOPort  Port=3  Side=Left
  Line A : PMIOPort  Port=4  Side=Right
  Line B : PMIOPort  Port=5  Side=Right
  Line C : PMIOPort  Port=6  Side=Right
  GAT A : PMIOPort  Port=7  Side=Right
  GAT B : PMIOPort  Port=8  Side=Right
  GAT C : PMIOPort  Port=9  Side=Right
  tag scope: P6_busIn_I=global, P6_busIn_V=global, P6_busOut_I=global, P6_busOut_V=global, P6_faultGIS_I=global, P6_faultGIS_V=global, P6_gatHV_I=global, P6_gatHV_V=global
  wires:
  [P6_BR_Q0] -> GSUT breaker Q0/1
  Bus incoming CT/1 -> [P6_busIn_V]
  Bus incoming CT/2 -> [P6_busIn_I]
  Line feeder CT/1 -> [P6_busOut_V]
  Line feeder CT/2 -> [P6_busOut_I]
  GAT feeder CT/1 -> [P6_gatHV_V]
  GAT feeder CT/2 -> [P6_gatHV_I]
  GIS bus fault measurement/1 -> [P6_faultGIS_V]
  GIS bus fault measurement/2 -> [P6_faultGIS_I]
  connections:
  GSUT A/RConn1 -- GSUT breaker Q0/LConn1
  GSUT B/RConn1 -- GSUT breaker Q0/LConn2
  GSUT C/RConn1 -- GSUT breaker Q0/LConn3
  GSUT breaker Q0/RConn1 -- Bus incoming CT/LConn1
  GSUT breaker Q0/RConn2 -- Bus incoming CT/LConn2
  GSUT breaker Q0/RConn3 -- Bus incoming CT/LConn3
  Line feeder CT/LConn1 -- Bus incoming CT/RConn1 -- GAT feeder CT/LConn1 -- GIS bus fault measurement/LConn1
  Line feeder CT/LConn2 -- Bus incoming CT/RConn2 -- GAT feeder CT/LConn2 -- GIS bus fault measurement/LConn2
  Line feeder CT/LConn3 -- Bus incoming CT/RConn3 -- GAT feeder CT/LConn3 -- GIS bus fault measurement/LConn3
  Line feeder CT/RConn1 -- Line A/RConn1
  Line feeder CT/RConn2 -- Line B/RConn1
  Line feeder CT/RConn3 -- Line C/RConn1
  GAT feeder CT/RConn1 -- GAT A/RConn1
  GAT feeder CT/RConn2 -- GAT B/RConn1
  GAT feeder CT/RConn3 -- GAT C/RConn1
  GIS bus fault measurement/RConn1 -- GIS bus fault/LConn1
  GIS bus fault measurement/RConn2 -- GIS bus fault/LConn2
  GIS bus fault measurement/RConn3 -- GIS bus fault/LConn3

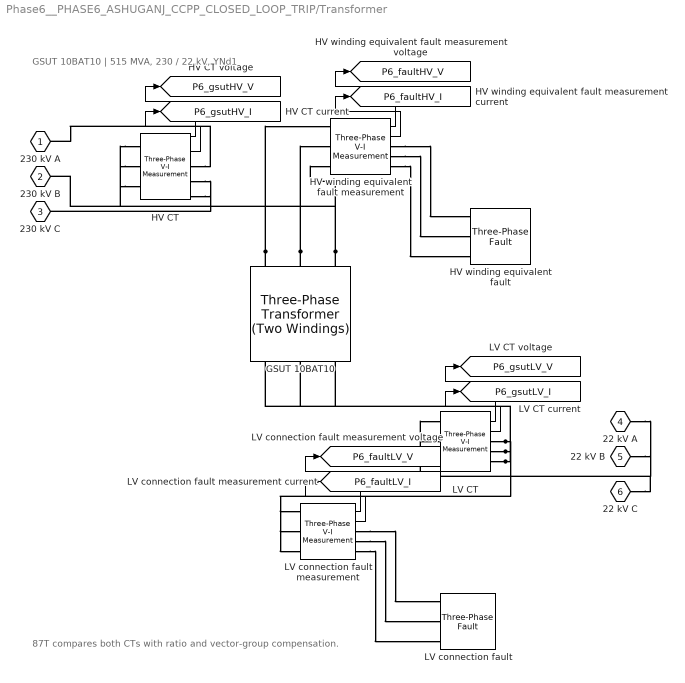
== system Phase6__PHASE6_ASHUGANJ_CCPP_CLOSED_LOOP_TRIP/Transformer ==
  note: GSUT 10BAT10 | 515 MVA, 230 / 22 kV, YNd1
  note: 87T compares both CTs with ratio and vector-group compensation.
  GSUT 10BAT10 : spsThreePhaseTransformerTwoWindingsLib/Three-Phase Transformer (Two Windings)  Winding1Connection=Yg  Winding2Connection=Delta (D1)  CoreType=Three single-phase transformers  SetSaturation=off  Hysteresis=off  DataFile='hysteresis'  SetInitialFlux=off  Measurements=None  UNITS=pu  NominalPower=[515000000 50]  Winding1=[230000 0.00105 0.07999310907822]  Winding2=[22000 0.00105 0.07999310907822]  Rm=3238.99371069182  Lm=791.886792163546  L0=0.158  Saturation=[ 0,0 ; 0.0024,1.2 ; 1.0,1.52 ]  InitialFluxes=[ 0.8 , -0.8 , 0.7 ]  BreakLoop=off  DiscreteSolver=Trapezoidal iterative  DataType=off  TransfoNumber=1
  HV CT : spsThreePhaseVIMeasurementLib/Three-Phase V-I Measurement  VoltageMeasurement=phase-to-ground  SetLabelV=off  LabelV=Vabc  Vpu=off  VpuLL=off  CurrentMeasurement=yes  SetLabelI=off  LabelI=Iabc  Ipu=off  Pbase=100e6  Vbase=500e3  OutputType=Complex  PhasorSimulation=off  PSBequivalent=0
  HV winding equivalent fault : spsThreePhaseFaultLib/Three-Phase Fault  InitialStates=0  FaultA=on  FaultB=on  FaultC=on  GroundFault=off  SwitchTimes=[1000000 1000001]  External=off  SwitchStatus=NaN  FaultResistance=0.01  GroundResistance=0.01  SnubberResistance=1000000000  SnubberCapacitance=inf  Measurements=None
  HV winding equivalent fault measurement : spsThreePhaseVIMeasurementLib/Three-Phase V-I Measurement  VoltageMeasurement=phase-to-ground  SetLabelV=off  LabelV=Vabc  Vpu=off  VpuLL=off  CurrentMeasurement=yes  SetLabelI=off  LabelI=Iabc  Ipu=off  Pbase=100e6  Vbase=500e3  OutputType=Complex  PhasorSimulation=off  PSBequivalent=0
  LV CT : spsThreePhaseVIMeasurementLib/Three-Phase V-I Measurement  VoltageMeasurement=phase-to-ground  SetLabelV=off  LabelV=Vabc  Vpu=off  VpuLL=off  CurrentMeasurement=yes  SetLabelI=off  LabelI=Iabc  Ipu=off  Pbase=100e6  Vbase=500e3  OutputType=Complex  PhasorSimulation=off  PSBequivalent=0
  LV connection fault : spsThreePhaseFaultLib/Three-Phase Fault  InitialStates=0  FaultA=on  FaultB=on  FaultC=on  GroundFault=off  SwitchTimes=[1000000 1000001]  External=off  SwitchStatus=NaN  FaultResistance=0.01  GroundResistance=0.01  SnubberResistance=1000000000  SnubberCapacitance=inf  Measurements=None
  LV connection fault measurement : spsThreePhaseVIMeasurementLib/Three-Phase V-I Measurement  VoltageMeasurement=phase-to-ground  SetLabelV=off  LabelV=Vabc  Vpu=off  VpuLL=off  CurrentMeasurement=yes  SetLabelI=off  LabelI=Iabc  Ipu=off  Pbase=100e6  Vbase=500e3  OutputType=Complex  PhasorSimulation=off  PSBequivalent=0
  230 kV A : PMIOPort  Side=Left
  230 kV B : PMIOPort  Port=2  Side=Left
  230 kV C : PMIOPort  Port=3  Side=Left
  22 kV A : PMIOPort  Port=4  Side=Right
  22 kV B : PMIOPort  Port=5  Side=Right
  22 kV C : PMIOPort  Port=6  Side=Right
  tag scope: P6_faultHV_I=global, P6_faultHV_V=global, P6_faultLV_I=global, P6_faultLV_V=global, P6_gsutHV_I=global, P6_gsutHV_V=global, P6_gsutLV_I=global, P6_gsutLV_V=global
  wires:
  LV CT/1 -> [P6_gsutLV_V]
  LV CT/2 -> [P6_gsutLV_I]
  LV connection fault measurement/1 -> [P6_faultLV_V]
  LV connection fault measurement/2 -> [P6_faultLV_I]
  HV CT/1 -> [P6_gsutHV_V]
  HV CT/2 -> [P6_gsutHV_I]
  HV winding equivalent fault measurement/1 -> [P6_faultHV_V]
  HV winding equivalent fault measurement/2 -> [P6_faultHV_I]
  connections:
  22 kV A/RConn1 -- LV CT/LConn1
  22 kV B/RConn1 -- LV CT/LConn2
  22 kV C/RConn1 -- LV CT/LConn3
  GSUT 10BAT10/RConn1 -- LV CT/RConn1 -- LV connection fault measurement/LConn1
  GSUT 10BAT10/RConn2 -- LV CT/RConn2 -- LV connection fault measurement/LConn2
  GSUT 10BAT10/RConn3 -- LV CT/RConn3 -- LV connection fault measurement/LConn3
  LV connection fault measurement/RConn1 -- LV connection fault/LConn1
  LV connection fault measurement/RConn2 -- LV connection fault/LConn2
  LV connection fault measurement/RConn3 -- LV connection fault/LConn3
  HV CT/LConn1 -- GSUT 10BAT10/LConn1 -- HV winding equivalent fault measurement/LConn1
  HV CT/LConn2 -- GSUT 10BAT10/LConn2 -- HV winding equivalent fault measurement/LConn2
  HV CT/LConn3 -- GSUT 10BAT10/LConn3 -- HV winding equivalent fault measurement/LConn3
  HV winding equivalent fault measurement/RConn1 -- HV winding equivalent fault/LConn1
  HV winding equivalent fault measurement/RConn2 -- HV winding equivalent fault/LConn2
  HV winding equivalent fault measurement/RConn3 -- HV winding equivalent fault/LConn3
  HV CT/RConn1 -- 230 kV A/RConn1
  HV CT/RConn2 -- 230 kV B/RConn1
  HV CT/RConn3 -- 230 kV C/RConn1
